simulink model "robot_2015_floor"  (R2017b)
(part 4 of 139)

  Revolute21 : sm_lib/Joints/Revolute Joint  SenseConstraintForce=off  SenseConstraintForceX=off  SenseConstraintForceY=off  SenseConstraintForceZ=off  SenseConstraintTorque=off  SenseConstraintTorqueX=off  SenseConstraintTorqueY=off  SenseConstraintTorqueZ=off  SenseTotalForce=off  SenseTotalForceX=off  SenseTotalForceY=off  SenseTotalForceZ=off  SenseTotalTorque=off  SenseTotalTorqueX=off  SenseTotalTorqueY=off  SenseTotalTorqueZ=off  CompositeWrenchDir=FollowerOnBase  CompositeWrenchFrame=BaseFrame  EquilibriumPosition=0  EquilibriumPositionUnits=rad  SpringStiffness=0  SpringStiffnessUnits=N*m/rad  DampingCoefficient=0  DampingCoefficientUnits=N*m/(rad/s)  TorqueActuationMode=NoTorque  MotionActuationMode=ComputedMotion  SensePosition=off  SenseVelocity=off  SenseAcceleration=off  SenseTorqueForce=off  PositionTargetSpecify=on  PositionTargetPriority=Low  PositionTargetValue=smiData.RevoluteJoint(650).Rz.Pos  PositionTargetValueUnits=deg  VelocityTargetSpecify=off  VelocityTargetPriority=High  VelocityTargetValue=0  VelocityTargetValueUnits=deg/s
  Revolute210 : sm_lib/Joints/Revolute Joint  SenseConstraintForce=off  SenseConstraintForceX=off  SenseConstraintForceY=off  SenseConstraintForceZ=off  SenseConstraintTorque=off  SenseConstraintTorqueX=off  SenseConstraintTorqueY=off  SenseConstraintTorqueZ=off  SenseTotalForce=off  SenseTotalForceX=off  SenseTotalForceY=off  SenseTotalForceZ=off  SenseTotalTorque=off  SenseTotalTorqueX=off  SenseTotalTorqueY=off  SenseTotalTorqueZ=off  CompositeWrenchDir=FollowerOnBase  CompositeWrenchFrame=BaseFrame  EquilibriumPosition=0  EquilibriumPositionUnits=rad  SpringStiffness=0  SpringStiffnessUnits=N*m/rad  DampingCoefficient=0  DampingCoefficientUnits=N*m/(rad/s)  TorqueActuationMode=NoTorque  MotionActuationMode=ComputedMotion  SensePosition=off  SenseVelocity=off  SenseAcceleration=off  SenseTorqueForce=off  PositionTargetSpecify=on  PositionTargetPriority=Low  PositionTargetValue=smiData.RevoluteJoint(839).Rz.Pos  PositionTargetValueUnits=deg  VelocityTargetSpecify=off  VelocityTargetPriority=High  VelocityTargetValue=0  VelocityTargetValueUnits=deg/s
  Revolute211 : sm_lib/Joints/Revolute Joint  SenseConstraintForce=off  SenseConstraintForceX=off  SenseConstraintForceY=off  SenseConstraintForceZ=off  SenseConstraintTorque=off  SenseConstraintTorqueX=off  SenseConstraintTorqueY=off  SenseConstraintTorqueZ=off  SenseTotalForce=off  SenseTotalForceX=off  SenseTotalForceY=off  SenseTotalForceZ=off  SenseTotalTorque=off  SenseTotalTorqueX=off  SenseTotalTorqueY=off  SenseTotalTorqueZ=off  CompositeWrenchDir=FollowerOnBase  CompositeWrenchFrame=BaseFrame  EquilibriumPosition=0  EquilibriumPositionUnits=rad  SpringStiffness=0  SpringStiffnessUnits=N*m/rad  DampingCoefficient=0  DampingCoefficientUnits=N*m/(rad/s)  TorqueActuationMode=NoTorque  MotionActuationMode=ComputedMotion  SensePosition=off  SenseVelocity=off  SenseAcceleration=off  SenseTorqueForce=off  PositionTargetSpecify=on  PositionTargetPriority=Low  PositionTargetValue=smiData.RevoluteJoint(840).Rz.Pos  PositionTargetValueUnits=deg  VelocityTargetSpecify=off  VelocityTargetPriority=High  VelocityTargetValue=0  VelocityTargetValueUnits=deg/s
  Revolute22 : sm_lib/Joints/Revolute Joint  SenseConstraintForce=off  SenseConstraintForceX=off  SenseConstraintForceY=off  SenseConstraintForceZ=off  SenseConstraintTorque=off  SenseConstraintTorqueX=off  SenseConstraintTorqueY=off  SenseConstraintTorqueZ=off  SenseTotalForce=off  SenseTotalForceX=off  SenseTotalForceY=off  SenseTotalForceZ=off  SenseTotalTorque=off  SenseTotalTorqueX=off  SenseTotalTorqueY=off  SenseTotalTorqueZ=off  CompositeWrenchDir=FollowerOnBase  CompositeWrenchFrame=BaseFrame  EquilibriumPosition=0  EquilibriumPositionUnits=rad  SpringStiffness=0  SpringStiffnessUnits=N*m/rad  DampingCoefficient=0  DampingCoefficientUnits=N*m/(rad/s)  TorqueActuationMode=NoTorque  MotionActuationMode=ComputedMotion  SensePosition=off  SenseVelocity=off  SenseAcceleration=off  SenseTorqueForce=off  PositionTargetSpecify=on  PositionTargetPriority=Low  PositionTargetValue=smiData.RevoluteJoint(651).Rz.Pos  PositionTargetValueUnits=deg  VelocityTargetSpecify=off  VelocityTargetPriority=High  VelocityTargetValue=0  VelocityTargetValueUnits=deg/s
  Revolute23 : sm_lib/Joints/Revolute Joint  SenseConstraintForce=off  SenseConstraintForceX=off  SenseConstraintForceY=off  SenseConstraintForceZ=off  SenseConstraintTorque=off  SenseConstraintTorqueX=off  SenseConstraintTorqueY=off  SenseConstraintTorqueZ=off  SenseTotalForce=off  SenseTotalForceX=off  SenseTotalForceY=off  SenseTotalForceZ=off  SenseTotalTorque=off  SenseTotalTorqueX=off  SenseTotalTorqueY=off  SenseTotalTorqueZ=off  CompositeWrenchDir=FollowerOnBase  CompositeWrenchFrame=BaseFrame  EquilibriumPosition=0  EquilibriumPositionUnits=rad  SpringStiffness=0  SpringStiffnessUnits=N*m/rad  DampingCoefficient=0  DampingCoefficientUnits=N*m/(rad/s)  TorqueActuationMode=NoTorque  MotionActuationMode=ComputedMotion  SensePosition=off  SenseVelocity=off  SenseAcceleration=off  SenseTorqueForce=off  PositionTargetSpecify=on  PositionTargetPriority=Low  PositionTargetValue=smiData.RevoluteJoint(652).Rz.Pos  PositionTargetValueUnits=deg  VelocityTargetSpecify=off  VelocityTargetPriority=High  VelocityTargetValue=0  VelocityTargetValueUnits=deg/s
  Revolute24 : sm_lib/Joints/Revolute Joint  SenseConstraintForce=off  SenseConstraintForceX=off  SenseConstraintForceY=off  SenseConstraintForceZ=off  SenseConstraintTorque=off  SenseConstraintTorqueX=off  SenseConstraintTorqueY=off  SenseConstraintTorqueZ=off  SenseTotalForce=off  SenseTotalForceX=off  SenseTotalForceY=off  SenseTotalForceZ=off  SenseTotalTorque=off  SenseTotalTorqueX=off  SenseTotalTorqueY=off  SenseTotalTorqueZ=off  CompositeWrenchDir=FollowerOnBase  CompositeWrenchFrame=BaseFrame  EquilibriumPosition=0  EquilibriumPositionUnits=rad  SpringStiffness=0  SpringStiffnessUnits=N*m/rad  DampingCoefficient=0  DampingCoefficientUnits=N*m/(rad/s)  TorqueActuationMode=NoTorque  MotionActuationMode=ComputedMotion  SensePosition=off  SenseVelocity=off  SenseAcceleration=off  SenseTorqueForce=off  PositionTargetSpecify=on  PositionTargetPriority=Low  PositionTargetValue=smiData.RevoluteJoint(653).Rz.Pos  PositionTargetValueUnits=deg  VelocityTargetSpecify=off  VelocityTargetPriority=High  VelocityTargetValue=0  VelocityTargetValueUnits=deg/s
  Revolute25 : sm_lib/Joints/Revolute Joint  SenseConstraintForce=off  SenseConstraintForceX=off  SenseConstraintForceY=off  SenseConstraintForceZ=off  SenseConstraintTorque=off  SenseConstraintTorqueX=off  SenseConstraintTorqueY=off  SenseConstraintTorqueZ=off  SenseTotalForce=off  SenseTotalForceX=off  SenseTotalForceY=off  SenseTotalForceZ=off  SenseTotalTorque=off  SenseTotalTorqueX=off  SenseTotalTorqueY=off  SenseTotalTorqueZ=off  CompositeWrenchDir=FollowerOnBase  CompositeWrenchFrame=BaseFrame  EquilibriumPosition=0  EquilibriumPositionUnits=rad  SpringStiffness=0  SpringStiffnessUnits=N*m/rad  DampingCoefficient=0  DampingCoefficientUnits=N*m/(rad/s)  TorqueActuationMode=NoTorque  MotionActuationMode=ComputedMotion  SensePosition=off  SenseVelocity=off  SenseAcceleration=off  SenseTorqueForce=off  PositionTargetSpecify=on  PositionTargetPriority=Low  PositionTargetValue=smiData.RevoluteJoint(654).Rz.Pos  PositionTargetValueUnits=deg  VelocityTargetSpecify=off  VelocityTargetPriority=High  VelocityTargetValue=0  VelocityTargetValueUnits=deg/s
  Revolute26 : sm_lib/Joints/Revolute Joint  SenseConstraintForce=off  SenseConstraintForceX=off  SenseConstraintForceY=off  SenseConstraintForceZ=off  SenseConstraintTorque=off  SenseConstraintTorqueX=off  SenseConstraintTorqueY=off  SenseConstraintTorqueZ=off  SenseTotalForce=off  SenseTotalForceX=off  SenseTotalForceY=off  SenseTotalForceZ=off  SenseTotalTorque=off  SenseTotalTorqueX=off  SenseTotalTorqueY=off  SenseTotalTorqueZ=off  CompositeWrenchDir=FollowerOnBase  CompositeWrenchFrame=BaseFrame  EquilibriumPosition=0  EquilibriumPositionUnits=rad  SpringStiffness=0  SpringStiffnessUnits=N*m/rad  DampingCoefficient=0  DampingCoefficientUnits=N*m/(rad/s)  TorqueActuationMode=NoTorque  MotionActuationMode=ComputedMotion  SensePosition=off  SenseVelocity=off  SenseAcceleration=off  SenseTorqueForce=off  PositionTargetSpecify=on  PositionTargetPriority=Low  PositionTargetValue=smiData.RevoluteJoint(655).Rz.Pos  PositionTargetValueUnits=deg  VelocityTargetSpecify=off  VelocityTargetPriority=High  VelocityTargetValue=0  VelocityTargetValueUnits=deg/s
  Revolute27 : sm_lib/Joints/Revolute Joint  SenseConstraintForce=off  SenseConstraintForceX=off  SenseConstraintForceY=off  SenseConstraintForceZ=off  SenseConstraintTorque=off  SenseConstraintTorqueX=off  SenseConstraintTorqueY=off  SenseConstraintTorqueZ=off  SenseTotalForce=off  SenseTotalForceX=off  SenseTotalForceY=off  SenseTotalForceZ=off  SenseTotalTorque=off  SenseTotalTorqueX=off  SenseTotalTorqueY=off  SenseTotalTorqueZ=off  CompositeWrenchDir=FollowerOnBase  CompositeWrenchFrame=BaseFrame  EquilibriumPosition=0  EquilibriumPositionUnits=rad  SpringStiffness=0  SpringStiffnessUnits=N*m/rad  DampingCoefficient=0  DampingCoefficientUnits=N*m/(rad/s)  TorqueActuationMode=NoTorque  MotionActuationMode=ComputedMotion  SensePosition=off  SenseVelocity=off  SenseAcceleration=off  SenseTorqueForce=off  PositionTargetSpecify=on  PositionTargetPriority=Low  PositionTargetValue=smiData.RevoluteJoint(656).Rz.Pos  PositionTargetValueUnits=deg  VelocityTargetSpecify=off  VelocityTargetPriority=High  VelocityTargetValue=0  VelocityTargetValueUnits=deg/s
  Revolute28 : sm_lib/Joints/Revolute Joint  SenseConstraintForce=off  SenseConstraintForceX=off  SenseConstraintForceY=off  SenseConstraintForceZ=off  SenseConstraintTorque=off  SenseConstraintTorqueX=off  SenseConstraintTorqueY=off  SenseConstraintTorqueZ=off  SenseTotalForce=off  SenseTotalForceX=off  SenseTotalForceY=off  SenseTotalForceZ=off  SenseTotalTorque=off  SenseTotalTorqueX=off  SenseTotalTorqueY=off  SenseTotalTorqueZ=off  CompositeWrenchDir=FollowerOnBase  CompositeWrenchFrame=BaseFrame  EquilibriumPosition=0  EquilibriumPositionUnits=rad  SpringStiffness=0  SpringStiffnessUnits=N*m/rad  DampingCoefficient=0  DampingCoefficientUnits=N*m/(rad/s)  TorqueActuationMode=NoTorque  MotionActuationMode=ComputedMotion  SensePosition=off  SenseVelocity=off  SenseAcceleration=off  SenseTorqueForce=off  PositionTargetSpecify=on  PositionTargetPriority=Low  PositionTargetValue=smiData.RevoluteJoint(657).Rz.Pos  PositionTargetValueUnits=deg  VelocityTargetSpecify=off  VelocityTargetPriority=High  VelocityTargetValue=0  VelocityTargetValueUnits=deg/s
  Revolute29 : sm_lib/Joints/Revolute Joint  SenseConstraintForce=off  SenseConstraintForceX=off  SenseConstraintForceY=off  SenseConstraintForceZ=off  SenseConstraintTorque=off  SenseConstraintTorqueX=off  SenseConstraintTorqueY=off  SenseConstraintTorqueZ=off  SenseTotalForce=off  SenseTotalForceX=off  SenseTotalForceY=off  SenseTotalForceZ=off  SenseTotalTorque=off  SenseTotalTorqueX=off  SenseTotalTorqueY=off  SenseTotalTorqueZ=off  CompositeWrenchDir=FollowerOnBase  CompositeWrenchFrame=BaseFrame  EquilibriumPosition=0  EquilibriumPositionUnits=rad  SpringStiffness=0  SpringStiffnessUnits=N*m/rad  DampingCoefficient=0  DampingCoefficientUnits=N*m/(rad/s)  TorqueActuationMode=NoTorque  MotionActuationMode=ComputedMotion  SensePosition=off  SenseVelocity=off  SenseAcceleration=off  SenseTorqueForce=off  PositionTargetSpecify=on  PositionTargetPriority=Low  PositionTargetValue=smiData.RevoluteJoint(658).Rz.Pos  PositionTargetValueUnits=deg  VelocityTargetSpecify=off  VelocityTargetPriority=High  VelocityTargetValue=0  VelocityTargetValueUnits=deg/s
  Revolute3 : sm_lib/Joints/Revolute Joint  SenseConstraintForce=off  SenseConstraintForceX=off  SenseConstraintForceY=off  SenseConstraintForceZ=off  SenseConstraintTorque=off  SenseConstraintTorqueX=off  SenseConstraintTorqueY=off  SenseConstraintTorqueZ=off  SenseTotalForce=off  SenseTotalForceX=off  SenseTotalForceY=off  SenseTotalForceZ=off  SenseTotalTorque=off  SenseTotalTorqueX=off  SenseTotalTorqueY=off  SenseTotalTorqueZ=off  CompositeWrenchDir=FollowerOnBase  CompositeWrenchFrame=BaseFrame  EquilibriumPosition=0  EquilibriumPositionUnits=rad  SpringStiffness=0  SpringStiffnessUnits=N*m/rad  DampingCoefficient=0  DampingCoefficientUnits=N*m/(rad/s)  TorqueActuationMode=NoTorque  MotionActuationMode=ComputedMotion  SensePosition=off  SenseVelocity=off  SenseAcceleration=off  SenseTorqueForce=off  PositionTargetSpecify=on  PositionTargetPriority=Low  PositionTargetValue=smiData.RevoluteJoint(632).Rz.Pos  PositionTargetValueUnits=deg  VelocityTargetSpecify=off  VelocityTargetPriority=High  VelocityTargetValue=0  VelocityTargetValueUnits=deg/s
  Revolute30 : sm_lib/Joints/Revolute Joint  SenseConstraintForce=off  SenseConstraintForceX=off  SenseConstraintForceY=off  SenseConstraintForceZ=off  SenseConstraintTorque=off  SenseConstraintTorqueX=off  SenseConstraintTorqueY=off  SenseConstraintTorqueZ=off  SenseTotalForce=off  SenseTotalForceX=off  SenseTotalForceY=off  SenseTotalForceZ=off  SenseTotalTorque=off  SenseTotalTorqueX=off  SenseTotalTorqueY=off  SenseTotalTorqueZ=off  CompositeWrenchDir=FollowerOnBase  CompositeWrenchFrame=BaseFrame  EquilibriumPosition=0  EquilibriumPositionUnits=rad  SpringStiffness=0  SpringStiffnessUnits=N*m/rad  DampingCoefficient=0  DampingCoefficientUnits=N*m/(rad/s)  TorqueActuationMode=NoTorque  MotionActuationMode=ComputedMotion  SensePosition=off  SenseVelocity=off  SenseAcceleration=off  SenseTorqueForce=off  PositionTargetSpecify=on  PositionTargetPriority=Low  PositionTargetValue=smiData.RevoluteJoint(659).Rz.Pos  PositionTargetValueUnits=deg  VelocityTargetSpecify=off  VelocityTargetPriority=High  VelocityTargetValue=0  VelocityTargetValueUnits=deg/s
  Revolute31 : sm_lib/Joints/Revolute Joint  SenseConstraintForce=off  SenseConstraintForceX=off  SenseConstraintForceY=off  SenseConstraintForceZ=off  SenseConstraintTorque=off  SenseConstraintTorqueX=off  SenseConstraintTorqueY=off  SenseConstraintTorqueZ=off  SenseTotalForce=off  SenseTotalForceX=off  SenseTotalForceY=off  SenseTotalForceZ=off  SenseTotalTorque=off  SenseTotalTorqueX=off  SenseTotalTorqueY=off  SenseTotalTorqueZ=off  CompositeWrenchDir=FollowerOnBase  CompositeWrenchFrame=BaseFrame  EquilibriumPosition=0  EquilibriumPositionUnits=rad  SpringStiffness=0  SpringStiffnessUnits=N*m/rad  DampingCoefficient=0  DampingCoefficientUnits=N*m/(rad/s)  TorqueActuationMode=NoTorque  MotionActuationMode=ComputedMotion  SensePosition=off  SenseVelocity=off  SenseAcceleration=off  SenseTorqueForce=off  PositionTargetSpecify=on  PositionTargetPriority=Low  PositionTargetValue=smiData.RevoluteJoint(660).Rz.Pos  PositionTargetValueUnits=deg  VelocityTargetSpecify=off  VelocityTargetPriority=High  VelocityTargetValue=0  VelocityTargetValueUnits=deg/s
  Revolute32 : sm_lib/Joints/Revolute Joint  SenseConstraintForce=off  SenseConstraintForceX=off  SenseConstraintForceY=off  SenseConstraintForceZ=off  SenseConstraintTorque=off  SenseConstraintTorqueX=off  SenseConstraintTorqueY=off  SenseConstraintTorqueZ=off  SenseTotalForce=off  SenseTotalForceX=off  SenseTotalForceY=off  SenseTotalForceZ=off  SenseTotalTorque=off  SenseTotalTorqueX=off  SenseTotalTorqueY=off  SenseTotalTorqueZ=off  CompositeWrenchDir=FollowerOnBase  CompositeWrenchFrame=BaseFrame  EquilibriumPosition=0  EquilibriumPositionUnits=rad  SpringStiffness=0  SpringStiffnessUnits=N*m/rad  DampingCoefficient=0  DampingCoefficientUnits=N*m/(rad/s)  TorqueActuationMode=NoTorque  MotionActuationMode=ComputedMotion  SensePosition=off  SenseVelocity=off  SenseAcceleration=off  SenseTorqueForce=off  PositionTargetSpecify=on  PositionTargetPriority=Low  PositionTargetValue=smiData.RevoluteJoint(661).Rz.Pos  PositionTargetValueUnits=deg  VelocityTargetSpecify=off  VelocityTargetPriority=High  VelocityTargetValue=0  VelocityTargetValueUnits=deg/s
  Revolute33 : sm_lib/Joints/Revolute Joint  SenseConstraintForce=off  SenseConstraintForceX=off  SenseConstraintForceY=off  SenseConstraintForceZ=off  SenseConstraintTorque=off  SenseConstraintTorqueX=off  SenseConstraintTorqueY=off  SenseConstraintTorqueZ=off  SenseTotalForce=off  SenseTotalForceX=off  SenseTotalForceY=off  SenseTotalForceZ=off  SenseTotalTorque=off  SenseTotalTorqueX=off  SenseTotalTorqueY=off  SenseTotalTorqueZ=off  CompositeWrenchDir=FollowerOnBase  CompositeWrenchFrame=BaseFrame  EquilibriumPosition=0  EquilibriumPositionUnits=rad  SpringStiffness=0  SpringStiffnessUnits=N*m/rad  DampingCoefficient=0  DampingCoefficientUnits=N*m/(rad/s)  TorqueActuationMode=NoTorque  MotionActuationMode=ComputedMotion  SensePosition=off  SenseVelocity=off  SenseAcceleration=off  SenseTorqueForce=off  PositionTargetSpecify=on  PositionTargetPriority=Low  PositionTargetValue=smiData.RevoluteJoint(662).Rz.Pos  PositionTargetValueUnits=deg  VelocityTargetSpecify=off  VelocityTargetPriority=High  VelocityTargetValue=0  VelocityTargetValueUnits=deg/s
  Revolute34 : sm_lib/Joints/Revolute Joint  SenseConstraintForce=off  SenseConstraintForceX=off  SenseConstraintForceY=off  SenseConstraintForceZ=off  SenseConstraintTorque=off  SenseConstraintTorqueX=off  SenseConstraintTorqueY=off  SenseConstraintTorqueZ=off  SenseTotalForce=off  SenseTotalForceX=off  SenseTotalForceY=off  SenseTotalForceZ=off  SenseTotalTorque=off  SenseTotalTorqueX=off  SenseTotalTorqueY=off  SenseTotalTorqueZ=off  CompositeWrenchDir=FollowerOnBase  CompositeWrenchFrame=BaseFrame  EquilibriumPosition=0  EquilibriumPositionUnits=rad  SpringStiffness=0  SpringStiffnessUnits=N*m/rad  DampingCoefficient=0  DampingCoefficientUnits=N*m/(rad/s)  TorqueActuationMode=NoTorque  MotionActuationMode=ComputedMotion  SensePosition=off  SenseVelocity=off  SenseAcceleration=off  SenseTorqueForce=off  PositionTargetSpecify=on  PositionTargetPriority=Low  PositionTargetValue=smiData.RevoluteJoint(663).Rz.Pos  PositionTargetValueUnits=deg  VelocityTargetSpecify=off  VelocityTargetPriority=High  VelocityTargetValue=0  VelocityTargetValueUnits=deg/s
  Revolute35 : sm_lib/Joints/Revolute Joint  SenseConstraintForce=off  SenseConstraintForceX=off  SenseConstraintForceY=off  SenseConstraintForceZ=off  SenseConstraintTorque=off  SenseConstraintTorqueX=off  SenseConstraintTorqueY=off  SenseConstraintTorqueZ=off  SenseTotalForce=off  SenseTotalForceX=off  SenseTotalForceY=off  SenseTotalForceZ=off  SenseTotalTorque=off  SenseTotalTorqueX=off  SenseTotalTorqueY=off  SenseTotalTorqueZ=off  CompositeWrenchDir=FollowerOnBase  CompositeWrenchFrame=BaseFrame  EquilibriumPosition=0  EquilibriumPositionUnits=rad  SpringStiffness=0  SpringStiffnessUnits=N*m/rad  DampingCoefficient=0  DampingCoefficientUnits=N*m/(rad/s)  TorqueActuationMode=NoTorque  MotionActuationMode=ComputedMotion  SensePosition=off  SenseVelocity=off  SenseAcceleration=off  SenseTorqueForce=off  PositionTargetSpecify=on  PositionTargetPriority=Low  PositionTargetValue=smiData.RevoluteJoint(664).Rz.Pos  PositionTargetValueUnits=deg  VelocityTargetSpecify=off  VelocityTargetPriority=High  VelocityTargetValue=0  VelocityTargetValueUnits=deg/s
  Revolute36 : sm_lib/Joints/Revolute Joint  SenseConstraintForce=off  SenseConstraintForceX=off  SenseConstraintForceY=off  SenseConstraintForceZ=off  SenseConstraintTorque=off  SenseConstraintTorqueX=off  SenseConstraintTorqueY=off  SenseConstraintTorqueZ=off  SenseTotalForce=off  SenseTotalForceX=off  SenseTotalForceY=off  SenseTotalForceZ=off  SenseTotalTorque=off  SenseTotalTorqueX=off  SenseTotalTorqueY=off  SenseTotalTorqueZ=off  CompositeWrenchDir=FollowerOnBase  CompositeWrenchFrame=BaseFrame  EquilibriumPosition=0  EquilibriumPositionUnits=rad  SpringStiffness=0  SpringStiffnessUnits=N*m/rad  DampingCoefficient=0  DampingCoefficientUnits=N*m/(rad/s)  TorqueActuationMode=NoTorque  MotionActuationMode=ComputedMotion  SensePosition=off  SenseVelocity=off  SenseAcceleration=off  SenseTorqueForce=off  PositionTargetSpecify=on  PositionTargetPriority=Low  PositionTargetValue=smiData.RevoluteJoint(665).Rz.Pos  PositionTargetValueUnits=deg  VelocityTargetSpecify=off  VelocityTargetPriority=High  VelocityTargetValue=0  VelocityTargetValueUnits=deg/s
  Revolute37 : sm_lib/Joints/Revolute Joint  SenseConstraintForce=off  SenseConstraintForceX=off  SenseConstraintForceY=off  SenseConstraintForceZ=off  SenseConstraintTorque=off  SenseConstraintTorqueX=off  SenseConstraintTorqueY=off  SenseConstraintTorqueZ=off  SenseTotalForce=off  SenseTotalForceX=off  SenseTotalForceY=off  SenseTotalForceZ=off  SenseTotalTorque=off  SenseTotalTorqueX=off  SenseTotalTorqueY=off  SenseTotalTorqueZ=off  CompositeWrenchDir=FollowerOnBase  CompositeWrenchFrame=BaseFrame  EquilibriumPosition=0  EquilibriumPositionUnits=rad  SpringStiffness=0  SpringStiffnessUnits=N*m/rad  DampingCoefficient=0  DampingCoefficientUnits=N*m/(rad/s)  TorqueActuationMode=NoTorque  MotionActuationMode=ComputedMotion  SensePosition=off  SenseVelocity=off  SenseAcceleration=off  SenseTorqueForce=off  PositionTargetSpecify=on  PositionTargetPriority=Low  PositionTargetValue=smiData.RevoluteJoint(666).Rz.Pos  PositionTargetValueUnits=deg  VelocityTargetSpecify=off  VelocityTargetPriority=High  VelocityTargetValue=0  VelocityTargetValueUnits=deg/s
  Revolute38 : sm_lib/Joints/Revolute Joint  SenseConstraintForce=off  SenseConstraintForceX=off  SenseConstraintForceY=off  SenseConstraintForceZ=off  SenseConstraintTorque=off  SenseConstraintTorqueX=off  SenseConstraintTorqueY=off  SenseConstraintTorqueZ=off  SenseTotalForce=off  SenseTotalForceX=off  SenseTotalForceY=off  SenseTotalForceZ=off  SenseTotalTorque=off  SenseTotalTorqueX=off  SenseTotalTorqueY=off  SenseTotalTorqueZ=off  CompositeWrenchDir=FollowerOnBase  CompositeWrenchFrame=BaseFrame  EquilibriumPosition=0  EquilibriumPositionUnits=rad  SpringStiffness=0  SpringStiffnessUnits=N*m/rad  DampingCoefficient=0  DampingCoefficientUnits=N*m/(rad/s)  TorqueActuationMode=NoTorque  MotionActuationMode=ComputedMotion  SensePosition=off  SenseVelocity=off  SenseAcceleration=off  SenseTorqueForce=off  PositionTargetSpecify=on  PositionTargetPriority=Low  PositionTargetValue=smiData.RevoluteJoint(667).Rz.Pos  PositionTargetValueUnits=deg  VelocityTargetSpecify=off  VelocityTargetPriority=High  VelocityTargetValue=0  VelocityTargetValueUnits=deg/s
  Revolute39 : sm_lib/Joints/Revolute Joint  SenseConstraintForce=off  SenseConstraintForceX=off  SenseConstraintForceY=off  SenseConstraintForceZ=off  SenseConstraintTorque=off  SenseConstraintTorqueX=off  SenseConstraintTorqueY=off  SenseConstraintTorqueZ=off  SenseTotalForce=off  SenseTotalForceX=off  SenseTotalForceY=off  SenseTotalForceZ=off  SenseTotalTorque=off  SenseTotalTorqueX=off  SenseTotalTorqueY=off  SenseTotalTorqueZ=off  CompositeWrenchDir=FollowerOnBase  CompositeWrenchFrame=BaseFrame  EquilibriumPosition=0  EquilibriumPositionUnits=rad  SpringStiffness=0  SpringStiffnessUnits=N*m/rad  DampingCoefficient=0  DampingCoefficientUnits=N*m/(rad/s)  TorqueActuationMode=NoTorque  MotionActuationMode=ComputedMotion  SensePosition=off  SenseVelocity=off  SenseAcceleration=off  SenseTorqueForce=off  PositionTargetSpecify=on  PositionTargetPriority=Low  PositionTargetValue=smiData.RevoluteJoint(668).Rz.Pos  PositionTargetValueUnits=deg  VelocityTargetSpecify=off  VelocityTargetPriority=High  VelocityTargetValue=0  VelocityTargetValueUnits=deg/s
  Revolute4 : sm_lib/Joints/Revolute Joint  SenseConstraintForce=off  SenseConstraintForceX=off  SenseConstraintForceY=off  SenseConstraintForceZ=off  SenseConstraintTorque=off  SenseConstraintTorqueX=off  SenseConstraintTorqueY=off  SenseConstraintTorqueZ=off  SenseTotalForce=off  SenseTotalForceX=off  SenseTotalForceY=off  SenseTotalForceZ=off  SenseTotalTorque=off  SenseTotalTorqueX=off  SenseTotalTorqueY=off  SenseTotalTorqueZ=off  CompositeWrenchDir=FollowerOnBase  CompositeWrenchFrame=BaseFrame  EquilibriumPosition=0  EquilibriumPositionUnits=rad  SpringStiffness=0  SpringStiffnessUnits=N*m/rad  DampingCoefficient=0  DampingCoefficientUnits=N*m/(rad/s)  TorqueActuationMode=NoTorque  MotionActuationMode=ComputedMotion  SensePosition=off  SenseVelocity=off  SenseAcceleration=off  SenseTorqueForce=off  PositionTargetSpecify=on  PositionTargetPriority=Low  PositionTargetValue=smiData.RevoluteJoint(633).Rz.Pos  PositionTargetValueUnits=deg  VelocityTargetSpecify=off  VelocityTargetPriority=High  VelocityTargetValue=0  VelocityTargetValueUnits=deg/s
  Revolute40 : sm_lib/Joints/Revolute Joint  SenseConstraintForce=off  SenseConstraintForceX=off  SenseConstraintForceY=off  SenseConstraintForceZ=off  SenseConstraintTorque=off  SenseConstraintTorqueX=off  SenseConstraintTorqueY=off  SenseConstraintTorqueZ=off  SenseTotalForce=off  SenseTotalForceX=off  SenseTotalForceY=off  SenseTotalForceZ=off  SenseTotalTorque=off  SenseTotalTorqueX=off  SenseTotalTorqueY=off  SenseTotalTorqueZ=off  CompositeWrenchDir=FollowerOnBase  CompositeWrenchFrame=BaseFrame  EquilibriumPosition=0  EquilibriumPositionUnits=rad  SpringStiffness=0  SpringStiffnessUnits=N*m/rad  DampingCoefficient=0  DampingCoefficientUnits=N*m/(rad/s)  TorqueActuationMode=NoTorque  MotionActuationMode=ComputedMotion  SensePosition=off  SenseVelocity=off  SenseAcceleration=off  SenseTorqueForce=off  PositionTargetSpecify=on  PositionTargetPriority=Low  PositionTargetValue=smiData.RevoluteJoint(669).Rz.Pos  PositionTargetValueUnits=deg  VelocityTargetSpecify=off  VelocityTargetPriority=High  VelocityTargetValue=0  VelocityTargetValueUnits=deg/s
  Revolute41 : sm_lib/Joints/Revolute Joint  SenseConstraintForce=off  SenseConstraintForceX=off  SenseConstraintForceY=off  SenseConstraintForceZ=off  SenseConstraintTorque=off  SenseConstraintTorqueX=off  SenseConstraintTorqueY=off  SenseConstraintTorqueZ=off  SenseTotalForce=off  SenseTotalForceX=off  SenseTotalForceY=off  SenseTotalForceZ=off  SenseTotalTorque=off  SenseTotalTorqueX=off  SenseTotalTorqueY=off  SenseTotalTorqueZ=off  CompositeWrenchDir=FollowerOnBase  CompositeWrenchFrame=BaseFrame  EquilibriumPosition=0  EquilibriumPositionUnits=rad  SpringStiffness=0  SpringStiffnessUnits=N*m/rad  DampingCoefficient=0  DampingCoefficientUnits=N*m/(rad/s)  TorqueActuationMode=NoTorque  MotionActuationMode=ComputedMotion  SensePosition=off  SenseVelocity=off  SenseAcceleration=off  SenseTorqueForce=off  PositionTargetSpecify=on  PositionTargetPriority=Low  PositionTargetValue=smiData.RevoluteJoint(670).Rz.Pos  PositionTargetValueUnits=deg  VelocityTargetSpecify=off  VelocityTargetPriority=High  VelocityTargetValue=0  VelocityTargetValueUnits=deg/s
  Revolute42 : sm_lib/Joints/Revolute Joint  SenseConstraintForce=off  SenseConstraintForceX=off  SenseConstraintForceY=off  SenseConstraintForceZ=off  SenseConstraintTorque=off  SenseConstraintTorqueX=off  SenseConstraintTorqueY=off  SenseConstraintTorqueZ=off  SenseTotalForce=off  SenseTotalForceX=off  SenseTotalForceY=off  SenseTotalForceZ=off  SenseTotalTorque=off  SenseTotalTorqueX=off  SenseTotalTorqueY=off  SenseTotalTorqueZ=off  CompositeWrenchDir=FollowerOnBase  CompositeWrenchFrame=BaseFrame  EquilibriumPosition=0  EquilibriumPositionUnits=rad  SpringStiffness=0  SpringStiffnessUnits=N*m/rad  DampingCoefficient=0  DampingCoefficientUnits=N*m/(rad/s)  TorqueActuationMode=NoTorque  MotionActuationMode=ComputedMotion  SensePosition=off  SenseVelocity=off  SenseAcceleration=off  SenseTorqueForce=off  PositionTargetSpecify=on  PositionTargetPriority=Low  PositionTargetValue=smiData.RevoluteJoint(671).Rz.Pos  PositionTargetValueUnits=deg  VelocityTargetSpecify=off  VelocityTargetPriority=High  VelocityTargetValue=0  VelocityTargetValueUnits=deg/s
  Revolute43 : sm_lib/Joints/Revolute Joint  SenseConstraintForce=off  SenseConstraintForceX=off  SenseConstraintForceY=off  SenseConstraintForceZ=off  SenseConstraintTorque=off  SenseConstraintTorqueX=off  SenseConstraintTorqueY=off  SenseConstraintTorqueZ=off  SenseTotalForce=off  SenseTotalForceX=off  SenseTotalForceY=off  SenseTotalForceZ=off  SenseTotalTorque=off  SenseTotalTorqueX=off  SenseTotalTorqueY=off  SenseTotalTorqueZ=off  CompositeWrenchDir=FollowerOnBase  CompositeWrenchFrame=BaseFrame  EquilibriumPosition=0  EquilibriumPositionUnits=rad  SpringStiffness=0  SpringStiffnessUnits=N*m/rad  DampingCoefficient=0  DampingCoefficientUnits=N*m/(rad/s)  TorqueActuationMode=NoTorque  MotionActuationMode=ComputedMotion  SensePosition=off  SenseVelocity=off  SenseAcceleration=off  SenseTorqueForce=off  PositionTargetSpecify=on  PositionTargetPriority=Low  PositionTargetValue=smiData.RevoluteJoint(672).Rz.Pos  PositionTargetValueUnits=deg  VelocityTargetSpecify=off  VelocityTargetPriority=High  VelocityTargetValue=0  VelocityTargetValueUnits=deg/s
  Revolute44 : sm_lib/Joints/Revolute Joint  SenseConstraintForce=off  SenseConstraintForceX=off  SenseConstraintForceY=off  SenseConstraintForceZ=off  SenseConstraintTorque=off  SenseConstraintTorqueX=off  SenseConstraintTorqueY=off  SenseConstraintTorqueZ=off  SenseTotalForce=off  SenseTotalForceX=off  SenseTotalForceY=off  SenseTotalForceZ=off  SenseTotalTorque=off  SenseTotalTorqueX=off  SenseTotalTorqueY=off  SenseTotalTorqueZ=off  CompositeWrenchDir=FollowerOnBase  CompositeWrenchFrame=BaseFrame  EquilibriumPosition=0  EquilibriumPositionUnits=rad  SpringStiffness=0  SpringStiffnessUnits=N*m/rad  DampingCoefficient=0  DampingCoefficientUnits=N*m/(rad/s)  TorqueActuationMode=NoTorque  MotionActuationMode=ComputedMotion  SensePosition=off  SenseVelocity=off  SenseAcceleration=off  SenseTorqueForce=off  PositionTargetSpecify=on  PositionTargetPriority=Low  PositionTargetValue=smiData.RevoluteJoint(673).Rz.Pos  PositionTargetValueUnits=deg  VelocityTargetSpecify=off  VelocityTargetPriority=High  VelocityTargetValue=0  VelocityTargetValueUnits=deg/s
  Revolute45 : sm_lib/Joints/Revolute Joint  SenseConstraintForce=off  SenseConstraintForceX=off  SenseConstraintForceY=off  SenseConstraintForceZ=off  SenseConstraintTorque=off  SenseConstraintTorqueX=off  SenseConstraintTorqueY=off  SenseConstraintTorqueZ=off  SenseTotalForce=off  SenseTotalForceX=off  SenseTotalForceY=off  SenseTotalForceZ=off  SenseTotalTorque=off  SenseTotalTorqueX=off  SenseTotalTorqueY=off  SenseTotalTorqueZ=off  CompositeWrenchDir=FollowerOnBase  CompositeWrenchFrame=BaseFrame  EquilibriumPosition=0  EquilibriumPositionUnits=rad  SpringStiffness=0  SpringStiffnessUnits=N*m/rad  DampingCoefficient=0  DampingCoefficientUnits=N*m/(rad/s)  TorqueActuationMode=NoTorque  MotionActuationMode=ComputedMotion  SensePosition=off  SenseVelocity=off  SenseAcceleration=off  SenseTorqueForce=off  PositionTargetSpecify=off  PositionTargetPriority=High  PositionTargetValue=0  PositionTargetValueUnits=deg  VelocityTargetSpecify=off  VelocityTargetPriority=High  VelocityTargetValue=0  VelocityTargetValueUnits=deg/s
  Revolute46 : sm_lib/Joints/Revolute Joint  SenseConstraintForce=off  SenseConstraintForceX=off  SenseConstraintForceY=off  SenseConstraintForceZ=off  SenseConstraintTorque=off  SenseConstraintTorqueX=off  SenseConstraintTorqueY=off  SenseConstraintTorqueZ=off  SenseTotalForce=off  SenseTotalForceX=off  SenseTotalForceY=off  SenseTotalForceZ=off  SenseTotalTorque=off  SenseTotalTorqueX=off  SenseTotalTorqueY=off  SenseTotalTorqueZ=off  CompositeWrenchDir=FollowerOnBase  CompositeWrenchFrame=BaseFrame  EquilibriumPosition=0  EquilibriumPositionUnits=rad  SpringStiffness=0  SpringStiffnessUnits=N*m/rad  DampingCoefficient=0  DampingCoefficientUnits=N*m/(rad/s)  TorqueActuationMode=NoTorque  MotionActuationMode=ComputedMotion  SensePosition=off  SenseVelocity=off  SenseAcceleration=off  SenseTorqueForce=off  PositionTargetSpecify=on  PositionTargetPriority=Low  PositionTargetValue=smiData.RevoluteJoint(675).Rz.Pos  PositionTargetValueUnits=deg  VelocityTargetSpecify=off  VelocityTargetPriority=High  VelocityTargetValue=0  VelocityTargetValueUnits=deg/s
  Revolute47 : sm_lib/Joints/Revolute Joint  SenseConstraintForce=off  SenseConstraintForceX=off  SenseConstraintForceY=off  SenseConstraintForceZ=off  SenseConstraintTorque=off  SenseConstraintTorqueX=off  SenseConstraintTorqueY=off  SenseConstraintTorqueZ=off  SenseTotalForce=off  SenseTotalForceX=off  SenseTotalForceY=off  SenseTotalForceZ=off  SenseTotalTorque=off  SenseTotalTorqueX=off  SenseTotalTorqueY=off  SenseTotalTorqueZ=off  CompositeWrenchDir=FollowerOnBase  CompositeWrenchFrame=BaseFrame  EquilibriumPosition=0  EquilibriumPositionUnits=rad  SpringStiffness=0  SpringStiffnessUnits=N*m/rad  DampingCoefficient=0  DampingCoefficientUnits=N*m/(rad/s)  TorqueActuationMode=InputTorque  MotionActuationMode=ComputedMotion  SensePosition=on  SenseVelocity=on  SenseAcceleration=off  SenseTorqueForce=off  PositionTargetSpecify=on  PositionTargetPriority=High  PositionTargetValue=3.14  PositionTargetValueUnits=rad  VelocityTargetSpecify=off  VelocityTargetPriority=High  VelocityTargetValue=0  VelocityTargetValueUnits=deg/s
  Revolute48 : sm_lib/Joints/Revolute Joint  SenseConstraintForce=off  SenseConstraintForceX=off  SenseConstraintForceY=off  SenseConstraintForceZ=off  SenseConstraintTorque=off  SenseConstraintTorqueX=off  SenseConstraintTorqueY=off  SenseConstraintTorqueZ=off  SenseTotalForce=off  SenseTotalForceX=off  SenseTotalForceY=off  SenseTotalForceZ=off  SenseTotalTorque=off  SenseTotalTorqueX=off  SenseTotalTorqueY=off  SenseTotalTorqueZ=off  CompositeWrenchDir=FollowerOnBase  CompositeWrenchFrame=BaseFrame  EquilibriumPosition=0  EquilibriumPositionUnits=rad  SpringStiffness=0  SpringStiffnessUnits=N*m/rad  DampingCoefficient=0  DampingCoefficientUnits=N*m/(rad/s)  TorqueActuationMode=InputTorque  MotionActuationMode=ComputedMotion  SensePosition=on  SenseVelocity=on  SenseAcceleration=off  SenseTorqueForce=off  PositionTargetSpecify=on  PositionTargetPriority=High  PositionTargetValue=-1  PositionTargetValueUnits=rad  VelocityTargetSpecify=off  VelocityTargetPriority=High  VelocityTargetValue=0  VelocityTargetValueUnits=deg/s
  Revolute49 : sm_lib/Joints/Revolute Joint  SenseConstraintForce=off  SenseConstraintForceX=off  SenseConstraintForceY=off  SenseConstraintForceZ=off  SenseConstraintTorque=off  SenseConstraintTorqueX=off  SenseConstraintTorqueY=off  SenseConstraintTorqueZ=off  SenseTotalForce=off  SenseTotalForceX=off  SenseTotalForceY=off  SenseTotalForceZ=off  SenseTotalTorque=off  SenseTotalTorqueX=off  SenseTotalTorqueY=off  SenseTotalTorqueZ=off  CompositeWrenchDir=FollowerOnBase  CompositeWrenchFrame=BaseFrame  EquilibriumPosition=0  EquilibriumPositionUnits=rad  SpringStiffness=0  SpringStiffnessUnits=N*m/rad  DampingCoefficient=0  DampingCoefficientUnits=N*m/(rad/s)  TorqueActuationMode=InputTorque  MotionActuationMode=ComputedMotion  SensePosition=on  SenseVelocity=on  SenseAcceleration=off  SenseTorqueForce=off  PositionTargetSpecify=on  PositionTargetPriority=High  PositionTargetValue=1.57  PositionTargetValueUnits=rad  VelocityTargetSpecify=off  VelocityTargetPriority=High  VelocityTargetValue=0  VelocityTargetValueUnits=deg/s
  Revolute5 : sm_lib/Joints/Revolute Joint  SenseConstraintForce=off  SenseConstraintForceX=off  SenseConstraintForceY=off  SenseConstraintForceZ=off  SenseConstraintTorque=off  SenseConstraintTorqueX=off  SenseConstraintTorqueY=off  SenseConstraintTorqueZ=off  SenseTotalForce=off  SenseTotalForceX=off  SenseTotalForceY=off  SenseTotalForceZ=off  SenseTotalTorque=off  SenseTotalTorqueX=off  SenseTotalTorqueY=off  SenseTotalTorqueZ=off  CompositeWrenchDir=FollowerOnBase  CompositeWrenchFrame=BaseFrame  EquilibriumPosition=0  EquilibriumPositionUnits=rad  SpringStiffness=0  SpringStiffnessUnits=N*m/rad  DampingCoefficient=0  DampingCoefficientUnits=N*m/(rad/s)  TorqueActuationMode=NoTorque  MotionActuationMode=ComputedMotion  SensePosition=off  SenseVelocity=off  SenseAcceleration=off  SenseTorqueForce=off  PositionTargetSpecify=on  PositionTargetPriority=Low  PositionTargetValue=smiData.RevoluteJoint(634).Rz.Pos  PositionTargetValueUnits=deg  VelocityTargetSpecify=off  VelocityTargetPriority=High  VelocityTargetValue=0  VelocityTargetValueUnits=deg/s
  Revolute50 : sm_lib/Joints/Revolute Joint  SenseConstraintForce=off  SenseConstraintForceX=off  SenseConstraintForceY=off  SenseConstraintForceZ=off  SenseConstraintTorque=off  SenseConstraintTorqueX=off  SenseConstraintTorqueY=off  SenseConstraintTorqueZ=off  SenseTotalForce=off  SenseTotalForceX=off  SenseTotalForceY=off  SenseTotalForceZ=off  SenseTotalTorque=off  SenseTotalTorqueX=off  SenseTotalTorqueY=off  SenseTotalTorqueZ=off  CompositeWrenchDir=FollowerOnBase  CompositeWrenchFrame=BaseFrame  EquilibriumPosition=0  EquilibriumPositionUnits=rad  SpringStiffness=0  SpringStiffnessUnits=N*m/rad  DampingCoefficient=0  DampingCoefficientUnits=N*m/(rad/s)  TorqueActuationMode=NoTorque  MotionActuationMode=ComputedMotion  SensePosition=off  SenseVelocity=off  SenseAcceleration=off  SenseTorqueForce=off  PositionTargetSpecify=on  PositionTargetPriority=Low  PositionTargetValue=smiData.RevoluteJoint(679).Rz.Pos  PositionTargetValueUnits=deg  VelocityTargetSpecify=off  VelocityTargetPriority=High  VelocityTargetValue=0  VelocityTargetValueUnits=deg/s
  Revolute51 : sm_lib/Joints/Revolute Joint  SenseConstraintForce=off  SenseConstraintForceX=off  SenseConstraintForceY=off  SenseConstraintForceZ=off  SenseConstraintTorque=off  SenseConstraintTorqueX=off  SenseConstraintTorqueY=off  SenseConstraintTorqueZ=off  SenseTotalForce=off  SenseTotalForceX=off  SenseTotalForceY=off  SenseTotalForceZ=off  SenseTotalTorque=off  SenseTotalTorqueX=off  SenseTotalTorqueY=off  SenseTotalTorqueZ=off  CompositeWrenchDir=FollowerOnBase  CompositeWrenchFrame=BaseFrame  EquilibriumPosition=0  EquilibriumPositionUnits=rad  SpringStiffness=0  SpringStiffnessUnits=N*m/rad  DampingCoefficient=0  DampingCoefficientUnits=N*m/(rad/s)  TorqueActuationMode=NoTorque  MotionActuationMode=ComputedMotion  SensePosition=off  SenseVelocity=off  SenseAcceleration=off  SenseTorqueForce=off  PositionTargetSpecify=on  PositionTargetPriority=Low  PositionTargetValue=smiData.RevoluteJoint(680).Rz.Pos  PositionTargetValueUnits=deg  VelocityTargetSpecify=off  VelocityTargetPriority=High  VelocityTargetValue=0  VelocityTargetValueUnits=deg/s
  Revolute52 : sm_lib/Joints/Revolute Joint  SenseConstraintForce=off  SenseConstraintForceX=off  SenseConstraintForceY=off  SenseConstraintForceZ=off  SenseConstraintTorque=off  SenseConstraintTorqueX=off  SenseConstraintTorqueY=off  SenseConstraintTorqueZ=off  SenseTotalForce=off  SenseTotalForceX=off  SenseTotalForceY=off  SenseTotalForceZ=off  SenseTotalTorque=off  SenseTotalTorqueX=off  SenseTotalTorqueY=off  SenseTotalTorqueZ=off  CompositeWrenchDir=FollowerOnBase  CompositeWrenchFrame=BaseFrame  EquilibriumPosition=0  EquilibriumPositionUnits=rad  SpringStiffness=0  SpringStiffnessUnits=N*m/rad  DampingCoefficient=0  DampingCoefficientUnits=N*m/(rad/s)  TorqueActuationMode=NoTorque  MotionActuationMode=ComputedMotion  SensePosition=off  SenseVelocity=off  SenseAcceleration=off  SenseTorqueForce=off  PositionTargetSpecify=on  PositionTargetPriority=Low  PositionTargetValue=smiData.RevoluteJoint(681).Rz.Pos  PositionTargetValueUnits=deg  VelocityTargetSpecify=off  VelocityTargetPriority=High  VelocityTargetValue=0  VelocityTargetValueUnits=deg/s
  Revolute53 : sm_lib/Joints/Revolute Joint  SenseConstraintForce=off  SenseConstraintForceX=off  SenseConstraintForceY=off  SenseConstraintForceZ=off  SenseConstraintTorque=off  SenseConstraintTorqueX=off  SenseConstraintTorqueY=off  SenseConstraintTorqueZ=off  SenseTotalForce=off  SenseTotalForceX=off  SenseTotalForceY=off  SenseTotalForceZ=off  SenseTotalTorque=off  SenseTotalTorqueX=off  SenseTotalTorqueY=off  SenseTotalTorqueZ=off  CompositeWrenchDir=FollowerOnBase  CompositeWrenchFrame=BaseFrame  EquilibriumPosition=0  EquilibriumPositionUnits=rad  SpringStiffness=0  SpringStiffnessUnits=N*m/rad  DampingCoefficient=0  DampingCoefficientUnits=N*m/(rad/s)  TorqueActuationMode=NoTorque  MotionActuationMode=ComputedMotion  SensePosition=off  SenseVelocity=off  SenseAcceleration=off  SenseTorqueForce=off  PositionTargetSpecify=on  PositionTargetPriority=Low  PositionTargetValue=smiData.RevoluteJoint(682).Rz.Pos  PositionTargetValueUnits=deg  VelocityTargetSpecify=off  VelocityTargetPriority=High  VelocityTargetValue=0  VelocityTargetValueUnits=deg/s
  Revolute54 : sm_lib/Joints/Revolute Joint  SenseConstraintForce=off  SenseConstraintForceX=off  SenseConstraintForceY=off  SenseConstraintForceZ=off  SenseConstraintTorque=off  SenseConstraintTorqueX=off  SenseConstraintTorqueY=off  SenseConstraintTorqueZ=off  SenseTotalForce=off  SenseTotalForceX=off  SenseTotalForceY=off  SenseTotalForceZ=off  SenseTotalTorque=off  SenseTotalTorqueX=off  SenseTotalTorqueY=off  SenseTotalTorqueZ=off  CompositeWrenchDir=FollowerOnBase  CompositeWrenchFrame=BaseFrame  EquilibriumPosition=0  EquilibriumPositionUnits=rad  SpringStiffness=0  SpringStiffnessUnits=N*m/rad  DampingCoefficient=0  DampingCoefficientUnits=N*m/(rad/s)  TorqueActuationMode=NoTorque  MotionActuationMode=ComputedMotion  SensePosition=off  SenseVelocity=off  SenseAcceleration=off  SenseTorqueForce=off  PositionTargetSpecify=on  PositionTargetPriority=Low  PositionTargetValue=smiData.RevoluteJoint(683).Rz.Pos  PositionTargetValueUnits=deg  VelocityTargetSpecify=off  VelocityTargetPriority=High  VelocityTargetValue=0  VelocityTargetValueUnits=deg/s
  Revolute55 : sm_lib/Joints/Revolute Joint  SenseConstraintForce=off  SenseConstraintForceX=off  SenseConstraintForceY=off  SenseConstraintForceZ=off  SenseConstraintTorque=off  SenseConstraintTorqueX=off  SenseConstraintTorqueY=off  SenseConstraintTorqueZ=off  SenseTotalForce=off  SenseTotalForceX=off  SenseTotalForceY=off  SenseTotalForceZ=off  SenseTotalTorque=off  SenseTotalTorqueX=off  SenseTotalTorqueY=off  SenseTotalTorqueZ=off  CompositeWrenchDir=FollowerOnBase  CompositeWrenchFrame=BaseFrame  EquilibriumPosition=0  EquilibriumPositionUnits=rad  SpringStiffness=0  SpringStiffnessUnits=N*m/rad  DampingCoefficient=0  DampingCoefficientUnits=N*m/(rad/s)  TorqueActuationMode=NoTorque  MotionActuationMode=ComputedMotion  SensePosition=off  SenseVelocity=off  SenseAcceleration=off  SenseTorqueForce=off  PositionTargetSpecify=on  PositionTargetPriority=Low  PositionTargetValue=smiData.RevoluteJoint(684).Rz.Pos  PositionTargetValueUnits=deg  VelocityTargetSpecify=off  VelocityTargetPriority=High  VelocityTargetValue=0  VelocityTargetValueUnits=deg/s
  Revolute56 : sm_lib/Joints/Revolute Joint  SenseConstraintForce=off  SenseConstraintForceX=off  SenseConstraintForceY=off  SenseConstraintForceZ=off  SenseConstraintTorque=off  SenseConstraintTorqueX=off  SenseConstraintTorqueY=off  SenseConstraintTorqueZ=off  SenseTotalForce=off  SenseTotalForceX=off  SenseTotalForceY=off  SenseTotalForceZ=off  SenseTotalTorque=off  SenseTotalTorqueX=off  SenseTotalTorqueY=off  SenseTotalTorqueZ=off  CompositeWrenchDir=FollowerOnBase  CompositeWrenchFrame=BaseFrame  EquilibriumPosition=0  EquilibriumPositionUnits=rad  SpringStiffness=0  SpringStiffnessUnits=N*m/rad  DampingCoefficient=0  DampingCoefficientUnits=N*m/(rad/s)  TorqueActuationMode=NoTorque  MotionActuationMode=ComputedMotion  SensePosition=off  SenseVelocity=off  SenseAcceleration=off  SenseTorqueForce=off  PositionTargetSpecify=on  PositionTargetPriority=Low  PositionTargetValue=smiData.RevoluteJoint(685).Rz.Pos  PositionTargetValueUnits=deg  VelocityTargetSpecify=off  VelocityTargetPriority=High  VelocityTargetValue=0  VelocityTargetValueUnits=deg/s
  Revolute57 : sm_lib/Joints/Revolute Joint  SenseConstraintForce=off  SenseConstraintForceX=off  SenseConstraintForceY=off  SenseConstraintForceZ=off  SenseConstraintTorque=off  SenseConstraintTorqueX=off  SenseConstraintTorqueY=off  SenseConstraintTorqueZ=off  SenseTotalForce=off  SenseTotalForceX=off  SenseTotalForceY=off  SenseTotalForceZ=off  SenseTotalTorque=off  SenseTotalTorqueX=off  SenseTotalTorqueY=off  SenseTotalTorqueZ=off  CompositeWrenchDir=FollowerOnBase  CompositeWrenchFrame=BaseFrame  EquilibriumPosition=0  EquilibriumPositionUnits=rad  SpringStiffness=0  SpringStiffnessUnits=N*m/rad  DampingCoefficient=0  DampingCoefficientUnits=N*m/(rad/s)  TorqueActuationMode=NoTorque  MotionActuationMode=ComputedMotion  SensePosition=off  SenseVelocity=off  SenseAcceleration=off  SenseTorqueForce=off  PositionTargetSpecify=off  PositionTargetPriority=High  PositionTargetValue=0  PositionTargetValueUnits=deg  VelocityTargetSpecify=off  VelocityTargetPriority=High  VelocityTargetValue=0  VelocityTargetValueUnits=deg/s
  Revolute58 : sm_lib/Joints/Revolute Joint  SenseConstraintForce=off  SenseConstraintForceX=off  SenseConstraintForceY=off  SenseConstraintForceZ=off  SenseConstraintTorque=off  SenseConstraintTorqueX=off  SenseConstraintTorqueY=off  SenseConstraintTorqueZ=off  SenseTotalForce=off  SenseTotalForceX=off  SenseTotalForceY=off  SenseTotalForceZ=off  SenseTotalTorque=off  SenseTotalTorqueX=off  SenseTotalTorqueY=off  SenseTotalTorqueZ=off  CompositeWrenchDir=FollowerOnBase  CompositeWrenchFrame=BaseFrame  EquilibriumPosition=0  EquilibriumPositionUnits=rad  SpringStiffness=0  SpringStiffnessUnits=N*m/rad  DampingCoefficient=0  DampingCoefficientUnits=N*m/(rad/s)  TorqueActuationMode=NoTorque  MotionActuationMode=ComputedMotion  SensePosition=off  SenseVelocity=off  SenseAcceleration=off  SenseTorqueForce=off  PositionTargetSpecify=on  PositionTargetPriority=Low  PositionTargetValue=smiData.RevoluteJoint(687).Rz.Pos  PositionTargetValueUnits=deg  VelocityTargetSpecify=off  VelocityTargetPriority=High  VelocityTargetValue=0  VelocityTargetValueUnits=deg/s
  Revolute59 : sm_lib/Joints/Revolute Joint  SenseConstraintForce=off  SenseConstraintForceX=off  SenseConstraintForceY=off  SenseConstraintForceZ=off  SenseConstraintTorque=off  SenseConstraintTorqueX=off  SenseConstraintTorqueY=off  SenseConstraintTorqueZ=off  SenseTotalForce=off  SenseTotalForceX=off  SenseTotalForceY=off  SenseTotalForceZ=off  SenseTotalTorque=off  SenseTotalTorqueX=off  SenseTotalTorqueY=off  SenseTotalTorqueZ=off  CompositeWrenchDir=FollowerOnBase  CompositeWrenchFrame=BaseFrame  EquilibriumPosition=0  EquilibriumPositionUnits=rad  SpringStiffness=0  SpringStiffnessUnits=N*m/rad  DampingCoefficient=0  DampingCoefficientUnits=N*m/(rad/s)  TorqueActuationMode=NoTorque  MotionActuationMode=ComputedMotion  SensePosition=off  SenseVelocity=off  SenseAcceleration=off  SenseTorqueForce=off  PositionTargetSpecify=on  PositionTargetPriority=Low  PositionTargetValue=smiData.RevoluteJoint(688).Rz.Pos  PositionTargetValueUnits=deg  VelocityTargetSpecify=off  VelocityTargetPriority=High  VelocityTargetValue=0  VelocityTargetValueUnits=deg/s
  Revolute6 : sm_lib/Joints/Revolute Joint  SenseConstraintForce=off  SenseConstraintForceX=off  SenseConstraintForceY=off  SenseConstraintForceZ=off  SenseConstraintTorque=off  SenseConstraintTorqueX=off  SenseConstraintTorqueY=off  SenseConstraintTorqueZ=off  SenseTotalForce=off  SenseTotalForceX=off  SenseTotalForceY=off  SenseTotalForceZ=off  SenseTotalTorque=off  SenseTotalTorqueX=off  SenseTotalTorqueY=off  SenseTotalTorqueZ=off  CompositeWrenchDir=FollowerOnBase  CompositeWrenchFrame=BaseFrame  EquilibriumPosition=0  EquilibriumPositionUnits=rad  SpringStiffness=0  SpringStiffnessUnits=N*m/rad  DampingCoefficient=0  DampingCoefficientUnits=N*m/(rad/s)  TorqueActuationMode=NoTorque  MotionActuationMode=ComputedMotion  SensePosition=off  SenseVelocity=off  SenseAcceleration=off  SenseTorqueForce=off  PositionTargetSpecify=on  PositionTargetPriority=Low  PositionTargetValue=smiData.RevoluteJoint(635).Rz.Pos  PositionTargetValueUnits=deg  VelocityTargetSpecify=off  VelocityTargetPriority=High  VelocityTargetValue=0  VelocityTargetValueUnits=deg/s
  Revolute60 : sm_lib/Joints/Revolute Joint  SenseConstraintForce=off  SenseConstraintForceX=off  SenseConstraintForceY=off  SenseConstraintForceZ=off  SenseConstraintTorque=off  SenseConstraintTorqueX=off  SenseConstraintTorqueY=off  SenseConstraintTorqueZ=off  SenseTotalForce=off  SenseTotalForceX=off  SenseTotalForceY=off  SenseTotalForceZ=off  SenseTotalTorque=off  SenseTotalTorqueX=off  SenseTotalTorqueY=off  SenseTotalTorqueZ=off  CompositeWrenchDir=FollowerOnBase  CompositeWrenchFrame=BaseFrame  EquilibriumPosition=0  EquilibriumPositionUnits=rad  SpringStiffness=0  SpringStiffnessUnits=N*m/rad  DampingCoefficient=0  DampingCoefficientUnits=N*m/(rad/s)  TorqueActuationMode=NoTorque  MotionActuationMode=ComputedMotion  SensePosition=off  SenseVelocity=off  SenseAcceleration=off  SenseTorqueForce=off  PositionTargetSpecify=on  PositionTargetPriority=Low  PositionTargetValue=smiData.RevoluteJoint(689).Rz.Pos  PositionTargetValueUnits=deg  VelocityTargetSpecify=off  VelocityTargetPriority=High  VelocityTargetValue=0  VelocityTargetValueUnits=deg/s
  Revolute61 : sm_lib/Joints/Revolute Joint  SenseConstraintForce=off  SenseConstraintForceX=off  SenseConstraintForceY=off  SenseConstraintForceZ=off  SenseConstraintTorque=off  SenseConstraintTorqueX=off  SenseConstraintTorqueY=off  SenseConstraintTorqueZ=off  SenseTotalForce=off  SenseTotalForceX=off  SenseTotalForceY=off  SenseTotalForceZ=off  SenseTotalTorque=off  SenseTotalTorqueX=off  SenseTotalTorqueY=off  SenseTotalTorqueZ=off  CompositeWrenchDir=FollowerOnBase  CompositeWrenchFrame=BaseFrame  EquilibriumPosition=0  EquilibriumPositionUnits=rad  SpringStiffness=0  SpringStiffnessUnits=N*m/rad  DampingCoefficient=0  DampingCoefficientUnits=N*m/(rad/s)  TorqueActuationMode=NoTorque  MotionActuationMode=ComputedMotion  SensePosition=off  SenseVelocity=off  SenseAcceleration=off  SenseTorqueForce=off  PositionTargetSpecify=on  PositionTargetPriority=Low  PositionTargetValue=smiData.RevoluteJoint(690).Rz.Pos  PositionTargetValueUnits=deg  VelocityTargetSpecify=off  VelocityTargetPriority=High  VelocityTargetValue=0  VelocityTargetValueUnits=deg/s
  Revolute62 : sm_lib/Joints/Revolute Joint  SenseConstraintForce=off  SenseConstraintForceX=off  SenseConstraintForceY=off  SenseConstraintForceZ=off  SenseConstraintTorque=off  SenseConstraintTorqueX=off  SenseConstraintTorqueY=off  SenseConstraintTorqueZ=off  SenseTotalForce=off  SenseTotalForceX=off  SenseTotalForceY=off  SenseTotalForceZ=off  SenseTotalTorque=off  SenseTotalTorqueX=off  SenseTotalTorqueY=off  SenseTotalTorqueZ=off  CompositeWrenchDir=FollowerOnBase  CompositeWrenchFrame=BaseFrame  EquilibriumPosition=0  EquilibriumPositionUnits=rad  SpringStiffness=0  SpringStiffnessUnits=N*m/rad  DampingCoefficient=0  DampingCoefficientUnits=N*m/(rad/s)  TorqueActuationMode=NoTorque  MotionActuationMode=ComputedMotion  SensePosition=off  SenseVelocity=off  SenseAcceleration=off  SenseTorqueForce=off  PositionTargetSpecify=on  PositionTargetPriority=Low  PositionTargetValue=smiData.RevoluteJoint(691).Rz.Pos  PositionTargetValueUnits=deg  VelocityTargetSpecify=off  VelocityTargetPriority=High  VelocityTargetValue=0  VelocityTargetValueUnits=deg/s
  Revolute63 : sm_lib/Joints/Revolute Joint  SenseConstraintForce=off  SenseConstraintForceX=off  SenseConstraintForceY=off  SenseConstraintForceZ=off  SenseConstraintTorque=off  SenseConstraintTorqueX=off  SenseConstraintTorqueY=off  SenseConstraintTorqueZ=off  SenseTotalForce=off  SenseTotalForceX=off  SenseTotalForceY=off  SenseTotalForceZ=off  SenseTotalTorque=off  SenseTotalTorqueX=off  SenseTotalTorqueY=off  SenseTotalTorqueZ=off  CompositeWrenchDir=FollowerOnBase  CompositeWrenchFrame=BaseFrame  EquilibriumPosition=0  EquilibriumPositionUnits=rad  SpringStiffness=0  SpringStiffnessUnits=N*m/rad  DampingCoefficient=0  DampingCoefficientUnits=N*m/(rad/s)  TorqueActuationMode=NoTorque  MotionActuationMode=ComputedMotion  SensePosition=off  SenseVelocity=off  SenseAcceleration=off  SenseTorqueForce=off  PositionTargetSpecify=on  PositionTargetPriority=Low  PositionTargetValue=smiData.RevoluteJoint(692).Rz.Pos  PositionTargetValueUnits=deg  VelocityTargetSpecify=off  VelocityTargetPriority=High  VelocityTargetValue=0  VelocityTargetValueUnits=deg/s
  Revolute64 : sm_lib/Joints/Revolute Joint  SenseConstraintForce=off  SenseConstraintForceX=off  SenseConstraintForceY=off  SenseConstraintForceZ=off  SenseConstraintTorque=off  SenseConstraintTorqueX=off  SenseConstraintTorqueY=off  SenseConstraintTorqueZ=off  SenseTotalForce=off  SenseTotalForceX=off  SenseTotalForceY=off  SenseTotalForceZ=off  SenseTotalTorque=off  SenseTotalTorqueX=off  SenseTotalTorqueY=off  SenseTotalTorqueZ=off  CompositeWrenchDir=FollowerOnBase  CompositeWrenchFrame=BaseFrame  EquilibriumPosition=0  EquilibriumPositionUnits=rad  SpringStiffness=0  SpringStiffnessUnits=N*m/rad  DampingCoefficient=0  DampingCoefficientUnits=N*m/(rad/s)  TorqueActuationMode=NoTorque  MotionActuationMode=ComputedMotion  SensePosition=off  SenseVelocity=off  SenseAcceleration=off  SenseTorqueForce=off  PositionTargetSpecify=on  PositionTargetPriority=Low  PositionTargetValue=smiData.RevoluteJoint(693).Rz.Pos  PositionTargetValueUnits=deg  VelocityTargetSpecify=off  VelocityTargetPriority=High  VelocityTargetValue=0  VelocityTargetValueUnits=deg/s
  Revolute65 : sm_lib/Joints/Revolute Joint  SenseConstraintForce=off  SenseConstraintForceX=off  SenseConstraintForceY=off  SenseConstraintForceZ=off  SenseConstraintTorque=off  SenseConstraintTorqueX=off  SenseConstraintTorqueY=off  SenseConstraintTorqueZ=off  SenseTotalForce=off  SenseTotalForceX=off  SenseTotalForceY=off  SenseTotalForceZ=off  SenseTotalTorque=off  SenseTotalTorqueX=off  SenseTotalTorqueY=off  SenseTotalTorqueZ=off  CompositeWrenchDir=FollowerOnBase  CompositeWrenchFrame=BaseFrame  EquilibriumPosition=0  EquilibriumPositionUnits=rad  SpringStiffness=0  SpringStiffnessUnits=N*m/rad  DampingCoefficient=0  DampingCoefficientUnits=N*m/(rad/s)  TorqueActuationMode=NoTorque  MotionActuationMode=ComputedMotion  SensePosition=off  SenseVelocity=off  SenseAcceleration=off  SenseTorqueForce=off  PositionTargetSpecify=on  PositionTargetPriority=Low  PositionTargetValue=smiData.RevoluteJoint(694).Rz.Pos  PositionTargetValueUnits=deg  VelocityTargetSpecify=off  VelocityTargetPriority=High  VelocityTargetValue=0  VelocityTargetValueUnits=deg/s
  Revolute66 : sm_lib/Joints/Revolute Joint  SenseConstraintForce=off  SenseConstraintForceX=off  SenseConstraintForceY=off  SenseConstraintForceZ=off  SenseConstraintTorque=off  SenseConstraintTorqueX=off  SenseConstraintTorqueY=off  SenseConstraintTorqueZ=off  SenseTotalForce=off  SenseTotalForceX=off  SenseTotalForceY=off  SenseTotalForceZ=off  SenseTotalTorque=off  SenseTotalTorqueX=off  SenseTotalTorqueY=off  SenseTotalTorqueZ=off  CompositeWrenchDir=FollowerOnBase  CompositeWrenchFrame=BaseFrame  EquilibriumPosition=0  EquilibriumPositionUnits=rad  SpringStiffness=0  SpringStiffnessUnits=N*m/rad  DampingCoefficient=0  DampingCoefficientUnits=N*m/(rad/s)  TorqueActuationMode=NoTorque  MotionActuationMode=ComputedMotion  SensePosition=off  SenseVelocity=off  SenseAcceleration=off  SenseTorqueForce=off  PositionTargetSpecify=on  PositionTargetPriority=Low  PositionTargetValue=smiData.RevoluteJoint(695).Rz.Pos  PositionTargetValueUnits=deg  VelocityTargetSpecify=off  VelocityTargetPriority=High  VelocityTargetValue=0  VelocityTargetValueUnits=deg/s
  Revolute67 : sm_lib/Joints/Revolute Joint  SenseConstraintForce=off  SenseConstraintForceX=off  SenseConstraintForceY=off  SenseConstraintForceZ=off  SenseConstraintTorque=off  SenseConstraintTorqueX=off  SenseConstraintTorqueY=off  SenseConstraintTorqueZ=off  SenseTotalForce=off  SenseTotalForceX=off  SenseTotalForceY=off  SenseTotalForceZ=off  SenseTotalTorque=off  SenseTotalTorqueX=off  SenseTotalTorqueY=off  SenseTotalTorqueZ=off  CompositeWrenchDir=FollowerOnBase  CompositeWrenchFrame=BaseFrame  EquilibriumPosition=0  EquilibriumPositionUnits=rad  SpringStiffness=0  SpringStiffnessUnits=N*m/rad  DampingCoefficient=0  DampingCoefficientUnits=N*m/(rad/s)  TorqueActuationMode=NoTorque  MotionActuationMode=ComputedMotion  SensePosition=off  SenseVelocity=off  SenseAcceleration=off  SenseTorqueForce=off  PositionTargetSpecify=on  PositionTargetPriority=Low  PositionTargetValue=smiData.RevoluteJoint(696).Rz.Pos  PositionTargetValueUnits=deg  VelocityTargetSpecify=off  VelocityTargetPriority=High  VelocityTargetValue=0  VelocityTargetValueUnits=deg/s
  Revolute68 : sm_lib/Joints/Revolute Joint  SenseConstraintForce=off  SenseConstraintForceX=off  SenseConstraintForceY=off  SenseConstraintForceZ=off  SenseConstraintTorque=off  SenseConstraintTorqueX=off  SenseConstraintTorqueY=off  SenseConstraintTorqueZ=off  SenseTotalForce=off  SenseTotalForceX=off  SenseTotalForceY=off  SenseTotalForceZ=off  SenseTotalTorque=off  SenseTotalTorqueX=off  SenseTotalTorqueY=off  SenseTotalTorqueZ=off  CompositeWrenchDir=FollowerOnBase  CompositeWrenchFrame=BaseFrame  EquilibriumPosition=0  EquilibriumPositionUnits=rad  SpringStiffness=0  SpringStiffnessUnits=N*m/rad  DampingCoefficient=0  DampingCoefficientUnits=N*m/(rad/s)  TorqueActuationMode=NoTorque  MotionActuationMode=ComputedMotion  SensePosition=off  SenseVelocity=off  SenseAcceleration=off  SenseTorqueForce=off  PositionTargetSpecify=on  PositionTargetPriority=Low  PositionTargetValue=smiData.RevoluteJoint(697).Rz.Pos  PositionTargetValueUnits=deg  VelocityTargetSpecify=off  VelocityTargetPriority=High  VelocityTargetValue=0  VelocityTargetValueUnits=deg/s
  Revolute69 : sm_lib/Joints/Revolute Joint  SenseConstraintForce=off  SenseConstraintForceX=off  SenseConstraintForceY=off  SenseConstraintForceZ=off  SenseConstraintTorque=off  SenseConstraintTorqueX=off  SenseConstraintTorqueY=off  SenseConstraintTorqueZ=off  SenseTotalForce=off  SenseTotalForceX=off  SenseTotalForceY=off  SenseTotalForceZ=off  SenseTotalTorque=off  SenseTotalTorqueX=off  SenseTotalTorqueY=off  SenseTotalTorqueZ=off  CompositeWrenchDir=FollowerOnBase  CompositeWrenchFrame=BaseFrame  EquilibriumPosition=0  EquilibriumPositionUnits=rad  SpringStiffness=0  SpringStiffnessUnits=N*m/rad  DampingCoefficient=0  DampingCoefficientUnits=N*m/(rad/s)  TorqueActuationMode=NoTorque  MotionActuationMode=ComputedMotion  SensePosition=off  SenseVelocity=off  SenseAcceleration=off  SenseTorqueForce=off  PositionTargetSpecify=on  PositionTargetPriority=Low  PositionTargetValue=smiData.RevoluteJoint(698).Rz.Pos  PositionTargetValueUnits=deg  VelocityTargetSpecify=off  VelocityTargetPriority=High  VelocityTargetValue=0  VelocityTargetValueUnits=deg/s
  Revolute7 : sm_lib/Joints/Revolute Joint  SenseConstraintForce=off  SenseConstraintForceX=off  SenseConstraintForceY=off  SenseConstraintForceZ=off  SenseConstraintTorque=off  SenseConstraintTorqueX=off  SenseConstraintTorqueY=off  SenseConstraintTorqueZ=off  SenseTotalForce=off  SenseTotalForceX=off  SenseTotalForceY=off  SenseTotalForceZ=off  SenseTotalTorque=off  SenseTotalTorqueX=off  SenseTotalTorqueY=off  SenseTotalTorqueZ=off  CompositeWrenchDir=FollowerOnBase  CompositeWrenchFrame=BaseFrame  EquilibriumPosition=0  EquilibriumPositionUnits=rad  SpringStiffness=0  SpringStiffnessUnits=N*m/rad  DampingCoefficient=0  DampingCoefficientUnits=N*m/(rad/s)  TorqueActuationMode=NoTorque  MotionActuationMode=ComputedMotion  SensePosition=off  SenseVelocity=off  SenseAcceleration=off  SenseTorqueForce=off  PositionTargetSpecify=on  PositionTargetPriority=Low  PositionTargetValue=smiData.RevoluteJoint(636).Rz.Pos  PositionTargetValueUnits=deg  VelocityTargetSpecify=off  VelocityTargetPriority=High  VelocityTargetValue=0  VelocityTargetValueUnits=deg/s
  Revolute70 : sm_lib/Joints/Revolute Joint  SenseConstraintForce=off  SenseConstraintForceX=off  SenseConstraintForceY=off  SenseConstraintForceZ=off  SenseConstraintTorque=off  SenseConstraintTorqueX=off  SenseConstraintTorqueY=off  SenseConstraintTorqueZ=off  SenseTotalForce=off  SenseTotalForceX=off  SenseTotalForceY=off  SenseTotalForceZ=off  SenseTotalTorque=off  SenseTotalTorqueX=off  SenseTotalTorqueY=off  SenseTotalTorqueZ=off  CompositeWrenchDir=FollowerOnBase  CompositeWrenchFrame=BaseFrame  EquilibriumPosition=0  EquilibriumPositionUnits=rad  SpringStiffness=0  SpringStiffnessUnits=N*m/rad  DampingCoefficient=0  DampingCoefficientUnits=N*m/(rad/s)  TorqueActuationMode=NoTorque  MotionActuationMode=ComputedMotion  SensePosition=off  SenseVelocity=off  SenseAcceleration=off  SenseTorqueForce=off  PositionTargetSpecify=on  PositionTargetPriority=Low  PositionTargetValue=smiData.RevoluteJoint(699).Rz.Pos  PositionTargetValueUnits=deg  VelocityTargetSpecify=off  VelocityTargetPriority=High  VelocityTargetValue=0  VelocityTargetValueUnits=deg/s
  Revolute71 : sm_lib/Joints/Revolute Joint  SenseConstraintForce=off  SenseConstraintForceX=off  SenseConstraintForceY=off  SenseConstraintForceZ=off  SenseConstraintTorque=off  SenseConstraintTorqueX=off  SenseConstraintTorqueY=off  SenseConstraintTorqueZ=off  SenseTotalForce=off  SenseTotalForceX=off  SenseTotalForceY=off  SenseTotalForceZ=off  SenseTotalTorque=off  SenseTotalTorqueX=off  SenseTotalTorqueY=off  SenseTotalTorqueZ=off  CompositeWrenchDir=FollowerOnBase  CompositeWrenchFrame=BaseFrame  EquilibriumPosition=0  EquilibriumPositionUnits=rad  SpringStiffness=0  SpringStiffnessUnits=N*m/rad  DampingCoefficient=0  DampingCoefficientUnits=N*m/(rad/s)  TorqueActuationMode=NoTorque  MotionActuationMode=ComputedMotion  SensePosition=off  SenseVelocity=off  SenseAcceleration=off  SenseTorqueForce=off  PositionTargetSpecify=on  PositionTargetPriority=Low  PositionTargetValue=smiData.RevoluteJoint(700).Rz.Pos  PositionTargetValueUnits=deg  VelocityTargetSpecify=off  VelocityTargetPriority=High  VelocityTargetValue=0  VelocityTargetValueUnits=deg/s
  Revolute72 : sm_lib/Joints/Revolute Joint  SenseConstraintForce=off  SenseConstraintForceX=off  SenseConstraintForceY=off  SenseConstraintForceZ=off  SenseConstraintTorque=off  SenseConstraintTorqueX=off  SenseConstraintTorqueY=off  SenseConstraintTorqueZ=off  SenseTotalForce=off  SenseTotalForceX=off  SenseTotalForceY=off  SenseTotalForceZ=off  SenseTotalTorque=off  SenseTotalTorqueX=off  SenseTotalTorqueY=off  SenseTotalTorqueZ=off  CompositeWrenchDir=FollowerOnBase  CompositeWrenchFrame=BaseFrame  EquilibriumPosition=0  EquilibriumPositionUnits=rad  SpringStiffness=0  SpringStiffnessUnits=N*m/rad  DampingCoefficient=0  DampingCoefficientUnits=N*m/(rad/s)  TorqueActuationMode=NoTorque  MotionActuationMode=ComputedMotion  SensePosition=off  SenseVelocity=off  SenseAcceleration=off  SenseTorqueForce=off  PositionTargetSpecify=on  PositionTargetPriority=Low  PositionTargetValue=smiData.RevoluteJoint(701).Rz.Pos  PositionTargetValueUnits=deg  VelocityTargetSpecify=off  VelocityTargetPriority=High  VelocityTargetValue=0  VelocityTargetValueUnits=deg/s
  Revolute73 : sm_lib/Joints/Revolute Joint  SenseConstraintForce=off  SenseConstraintForceX=off  SenseConstraintForceY=off  SenseConstraintForceZ=off  SenseConstraintTorque=off  SenseConstraintTorqueX=off  SenseConstraintTorqueY=off  SenseConstraintTorqueZ=off  SenseTotalForce=off  SenseTotalForceX=off  SenseTotalForceY=off  SenseTotalForceZ=off  SenseTotalTorque=off  SenseTotalTorqueX=off  SenseTotalTorqueY=off  SenseTotalTorqueZ=off  CompositeWrenchDir=FollowerOnBase  CompositeWrenchFrame=BaseFrame  EquilibriumPosition=0  EquilibriumPositionUnits=rad  SpringStiffness=0  SpringStiffnessUnits=N*m/rad  DampingCoefficient=0  DampingCoefficientUnits=N*m/(rad/s)  TorqueActuationMode=NoTorque  MotionActuationMode=ComputedMotion  SensePosition=off  SenseVelocity=off  SenseAcceleration=off  SenseTorqueForce=off  PositionTargetSpecify=on  PositionTargetPriority=Low  PositionTargetValue=smiData.RevoluteJoint(702).Rz.Pos  PositionTargetValueUnits=deg  VelocityTargetSpecify=off  VelocityTargetPriority=High  VelocityTargetValue=0  VelocityTargetValueUnits=deg/s
  Revolute74 : sm_lib/Joints/Revolute Joint  SenseConstraintForce=off  SenseConstraintForceX=off  SenseConstraintForceY=off  SenseConstraintForceZ=off  SenseConstraintTorque=off  SenseConstraintTorqueX=off  SenseConstraintTorqueY=off  SenseConstraintTorqueZ=off  SenseTotalForce=off  SenseTotalForceX=off  SenseTotalForceY=off  SenseTotalForceZ=off  SenseTotalTorque=off  SenseTotalTorqueX=off  SenseTotalTorqueY=off  SenseTotalTorqueZ=off  CompositeWrenchDir=FollowerOnBase  CompositeWrenchFrame=BaseFrame  EquilibriumPosition=0  EquilibriumPositionUnits=rad  SpringStiffness=0  SpringStiffnessUnits=N*m/rad  DampingCoefficient=0  DampingCoefficientUnits=N*m/(rad/s)  TorqueActuationMode=NoTorque  MotionActuationMode=ComputedMotion  SensePosition=off  SenseVelocity=off  SenseAcceleration=off  SenseTorqueForce=off  PositionTargetSpecify=on  PositionTargetPriority=Low  PositionTargetValue=smiData.RevoluteJoint(703).Rz.Pos  PositionTargetValueUnits=deg  VelocityTargetSpecify=off  VelocityTargetPriority=High  VelocityTargetValue=0  VelocityTargetValueUnits=deg/s
  Revolute75 : sm_lib/Joints/Revolute Joint  SenseConstraintForce=off  SenseConstraintForceX=off  SenseConstraintForceY=off  SenseConstraintForceZ=off  SenseConstraintTorque=off  SenseConstraintTorqueX=off  SenseConstraintTorqueY=off  SenseConstraintTorqueZ=off  SenseTotalForce=off  SenseTotalForceX=off  SenseTotalForceY=off  SenseTotalForceZ=off  SenseTotalTorque=off  SenseTotalTorqueX=off  SenseTotalTorqueY=off  SenseTotalTorqueZ=off  CompositeWrenchDir=FollowerOnBase  CompositeWrenchFrame=BaseFrame  EquilibriumPosition=0  EquilibriumPositionUnits=rad  SpringStiffness=0  SpringStiffnessUnits=N*m/rad  DampingCoefficient=0  DampingCoefficientUnits=N*m/(rad/s)  TorqueActuationMode=NoTorque  MotionActuationMode=ComputedMotion  SensePosition=off  SenseVelocity=off  SenseAcceleration=off  SenseTorqueForce=off  PositionTargetSpecify=on  PositionTargetPriority=Low  PositionTargetValue=smiData.RevoluteJoint(704).Rz.Pos  PositionTargetValueUnits=deg  VelocityTargetSpecify=off  VelocityTargetPriority=High  VelocityTargetValue=0  VelocityTargetValueUnits=deg/s
  Revolute76 : sm_lib/Joints/Revolute Joint  SenseConstraintForce=off  SenseConstraintForceX=off  SenseConstraintForceY=off  SenseConstraintForceZ=off  SenseConstraintTorque=off  SenseConstraintTorqueX=off  SenseConstraintTorqueY=off  SenseConstraintTorqueZ=off  SenseTotalForce=off  SenseTotalForceX=off  SenseTotalForceY=off  SenseTotalForceZ=off  SenseTotalTorque=off  SenseTotalTorqueX=off  SenseTotalTorqueY=off  SenseTotalTorqueZ=off  CompositeWrenchDir=FollowerOnBase  CompositeWrenchFrame=BaseFrame  EquilibriumPosition=0  EquilibriumPositionUnits=rad  SpringStiffness=0  SpringStiffnessUnits=N*m/rad  DampingCoefficient=0  DampingCoefficientUnits=N*m/(rad/s)  TorqueActuationMode=NoTorque  MotionActuationMode=ComputedMotion  SensePosition=off  SenseVelocity=off  SenseAcceleration=off  SenseTorqueForce=off  PositionTargetSpecify=on  PositionTargetPriority=Low  PositionTargetValue=smiData.RevoluteJoint(705).Rz.Pos  PositionTargetValueUnits=deg  VelocityTargetSpecify=off  VelocityTargetPriority=High  VelocityTargetValue=0  VelocityTargetValueUnits=deg/s
  Revolute77 : sm_lib/Joints/Revolute Joint  SenseConstraintForce=off  SenseConstraintForceX=off  SenseConstraintForceY=off  SenseConstraintForceZ=off  SenseConstraintTorque=off  SenseConstraintTorqueX=off  SenseConstraintTorqueY=off  SenseConstraintTorqueZ=off  SenseTotalForce=off  SenseTotalForceX=off  SenseTotalForceY=off  SenseTotalForceZ=off  SenseTotalTorque=off  SenseTotalTorqueX=off  SenseTotalTorqueY=off  SenseTotalTorqueZ=off  CompositeWrenchDir=FollowerOnBase  CompositeWrenchFrame=BaseFrame  EquilibriumPosition=0  EquilibriumPositionUnits=rad  SpringStiffness=0  SpringStiffnessUnits=N*m/rad  DampingCoefficient=0  DampingCoefficientUnits=N*m/(rad/s)  TorqueActuationMode=NoTorque  MotionActuationMode=ComputedMotion  SensePosition=off  SenseVelocity=off  SenseAcceleration=off  SenseTorqueForce=off  PositionTargetSpecify=on  PositionTargetPriority=Low  PositionTargetValue=smiData.RevoluteJoint(706).Rz.Pos  PositionTargetValueUnits=deg  VelocityTargetSpecify=off  VelocityTargetPriority=High  VelocityTargetValue=0  VelocityTargetValueUnits=deg/s
  Revolute78 : sm_lib/Joints/Revolute Joint  SenseConstraintForce=off  SenseConstraintForceX=off  SenseConstraintForceY=off  SenseConstraintForceZ=off  SenseConstraintTorque=off  SenseConstraintTorqueX=off  SenseConstraintTorqueY=off  SenseConstraintTorqueZ=off  SenseTotalForce=off  SenseTotalForceX=off  SenseTotalForceY=off  SenseTotalForceZ=off  SenseTotalTorque=off  SenseTotalTorqueX=off  SenseTotalTorqueY=off  SenseTotalTorqueZ=off  CompositeWrenchDir=FollowerOnBase  CompositeWrenchFrame=BaseFrame  EquilibriumPosition=0  EquilibriumPositionUnits=rad  SpringStiffness=0  SpringStiffnessUnits=N*m/rad  DampingCoefficient=0  DampingCoefficientUnits=N*m/(rad/s)  TorqueActuationMode=NoTorque  MotionActuationMode=ComputedMotion  SensePosition=off  SenseVelocity=off  SenseAcceleration=off  SenseTorqueForce=off  PositionTargetSpecify=on  PositionTargetPriority=Low  PositionTargetValue=smiData.RevoluteJoint(707).Rz.Pos  PositionTargetValueUnits=deg  VelocityTargetSpecify=off  VelocityTargetPriority=High  VelocityTargetValue=0  VelocityTargetValueUnits=deg/s
  Revolute79 : sm_lib/Joints/Revolute Joint  SenseConstraintForce=off  SenseConstraintForceX=off  SenseConstraintForceY=off  SenseConstraintForceZ=off  SenseConstraintTorque=off  SenseConstraintTorqueX=off  SenseConstraintTorqueY=off  SenseConstraintTorqueZ=off  SenseTotalForce=off  SenseTotalForceX=off  SenseTotalForceY=off  SenseTotalForceZ=off  SenseTotalTorque=off  SenseTotalTorqueX=off  SenseTotalTorqueY=off  SenseTotalTorqueZ=off  CompositeWrenchDir=FollowerOnBase  CompositeWrenchFrame=BaseFrame  EquilibriumPosition=0  EquilibriumPositionUnits=rad  SpringStiffness=0  SpringStiffnessUnits=N*m/rad  DampingCoefficient=0  DampingCoefficientUnits=N*m/(rad/s)  TorqueActuationMode=NoTorque  MotionActuationMode=ComputedMotion  SensePosition=off  SenseVelocity=off  SenseAcceleration=off  SenseTorqueForce=off  PositionTargetSpecify=on  PositionTargetPriority=Low  PositionTargetValue=smiData.RevoluteJoint(708).Rz.Pos  PositionTargetValueUnits=deg  VelocityTargetSpecify=off  VelocityTargetPriority=High  VelocityTargetValue=0  VelocityTargetValueUnits=deg/s
  Revolute8 : sm_lib/Joints/Revolute Joint  SenseConstraintForce=off  SenseConstraintForceX=off  SenseConstraintForceY=off  SenseConstraintForceZ=off  SenseConstraintTorque=off  SenseConstraintTorqueX=off  SenseConstraintTorqueY=off  SenseConstraintTorqueZ=off  SenseTotalForce=off  SenseTotalForceX=off  SenseTotalForceY=off  SenseTotalForceZ=off  SenseTotalTorque=off  SenseTotalTorqueX=off  SenseTotalTorqueY=off  SenseTotalTorqueZ=off  CompositeWrenchDir=FollowerOnBase  CompositeWrenchFrame=BaseFrame  EquilibriumPosition=0  EquilibriumPositionUnits=rad  SpringStiffness=0  SpringStiffnessUnits=N*m/rad  DampingCoefficient=0  DampingCoefficientUnits=N*m/(rad/s)  TorqueActuationMode=NoTorque  MotionActuationMode=ComputedMotion  SensePosition=off  SenseVelocity=off  SenseAcceleration=off  SenseTorqueForce=off  PositionTargetSpecify=on  PositionTargetPriority=Low  PositionTargetValue=smiData.RevoluteJoint(637).Rz.Pos  PositionTargetValueUnits=deg  VelocityTargetSpecify=off  VelocityTargetPriority=High  VelocityTargetValue=0  VelocityTargetValueUnits=deg/s
  Revolute80 : sm_lib/Joints/Revolute Joint  SenseConstraintForce=off  SenseConstraintForceX=off  SenseConstraintForceY=off  SenseConstraintForceZ=off  SenseConstraintTorque=off  SenseConstraintTorqueX=off  SenseConstraintTorqueY=off  SenseConstraintTorqueZ=off  SenseTotalForce=off  SenseTotalForceX=off  SenseTotalForceY=off  SenseTotalForceZ=off  SenseTotalTorque=off  SenseTotalTorqueX=off  SenseTotalTorqueY=off  SenseTotalTorqueZ=off  CompositeWrenchDir=FollowerOnBase  CompositeWrenchFrame=BaseFrame  EquilibriumPosition=0  EquilibriumPositionUnits=rad  SpringStiffness=0  SpringStiffnessUnits=N*m/rad  DampingCoefficient=0  DampingCoefficientUnits=N*m/(rad/s)  TorqueActuationMode=NoTorque  MotionActuationMode=ComputedMotion  SensePosition=off  SenseVelocity=off  SenseAcceleration=off  SenseTorqueForce=off  PositionTargetSpecify=on  PositionTargetPriority=Low  PositionTargetValue=smiData.RevoluteJoint(709).Rz.Pos  PositionTargetValueUnits=deg  VelocityTargetSpecify=off  VelocityTargetPriority=High  VelocityTargetValue=0  VelocityTargetValueUnits=deg/s
  Revolute81 : sm_lib/Joints/Revolute Joint  SenseConstraintForce=off  SenseConstraintForceX=off  SenseConstraintForceY=off  SenseConstraintForceZ=off  SenseConstraintTorque=off  SenseConstraintTorqueX=off  SenseConstraintTorqueY=off  SenseConstraintTorqueZ=off  SenseTotalForce=off  SenseTotalForceX=off  SenseTotalForceY=off  SenseTotalForceZ=off  SenseTotalTorque=off  SenseTotalTorqueX=off  SenseTotalTorqueY=off  SenseTotalTorqueZ=off  CompositeWrenchDir=FollowerOnBase  CompositeWrenchFrame=BaseFrame  EquilibriumPosition=0  EquilibriumPositionUnits=rad  SpringStiffness=0  SpringStiffnessUnits=N*m/rad  DampingCoefficient=0  DampingCoefficientUnits=N*m/(rad/s)  TorqueActuationMode=NoTorque  MotionActuationMode=ComputedMotion  SensePosition=off  SenseVelocity=off  SenseAcceleration=off  SenseTorqueForce=off  PositionTargetSpecify=on  PositionTargetPriority=Low  PositionTargetValue=smiData.RevoluteJoint(710).Rz.Pos  PositionTargetValueUnits=deg  VelocityTargetSpecify=off  VelocityTargetPriority=High  VelocityTargetValue=0  VelocityTargetValueUnits=deg/s
  Revolute82 : sm_lib/Joints/Revolute Joint  SenseConstraintForce=off  SenseConstraintForceX=off  SenseConstraintForceY=off  SenseConstraintForceZ=off  SenseConstraintTorque=off  SenseConstraintTorqueX=off  SenseConstraintTorqueY=off  SenseConstraintTorqueZ=off  SenseTotalForce=off  SenseTotalForceX=off  SenseTotalForceY=off  SenseTotalForceZ=off  SenseTotalTorque=off  SenseTotalTorqueX=off  SenseTotalTorqueY=off  SenseTotalTorqueZ=off  CompositeWrenchDir=FollowerOnBase  CompositeWrenchFrame=BaseFrame  EquilibriumPosition=0  EquilibriumPositionUnits=rad  SpringStiffness=0  SpringStiffnessUnits=N*m/rad  DampingCoefficient=0  DampingCoefficientUnits=N*m/(rad/s)  TorqueActuationMode=NoTorque  MotionActuationMode=ComputedMotion  SensePosition=off  SenseVelocity=off  SenseAcceleration=off  SenseTorqueForce=off  PositionTargetSpecify=on  PositionTargetPriority=Low  PositionTargetValue=smiData.RevoluteJoint(711).Rz.Pos  PositionTargetValueUnits=deg  VelocityTargetSpecify=off  VelocityTargetPriority=High  VelocityTargetValue=0  VelocityTargetValueUnits=deg/s
  Revolute83 : sm_lib/Joints/Revolute Joint  SenseConstraintForce=off  SenseConstraintForceX=off  SenseConstraintForceY=off  SenseConstraintForceZ=off  SenseConstraintTorque=off  SenseConstraintTorqueX=off  SenseConstraintTorqueY=off  SenseConstraintTorqueZ=off  SenseTotalForce=off  SenseTotalForceX=off  SenseTotalForceY=off  SenseTotalForceZ=off  SenseTotalTorque=off  SenseTotalTorqueX=off  SenseTotalTorqueY=off  SenseTotalTorqueZ=off  CompositeWrenchDir=FollowerOnBase  CompositeWrenchFrame=BaseFrame  EquilibriumPosition=0  EquilibriumPositionUnits=rad  SpringStiffness=0  SpringStiffnessUnits=N*m/rad  DampingCoefficient=0  DampingCoefficientUnits=N*m/(rad/s)  TorqueActuationMode=NoTorque  MotionActuationMode=ComputedMotion  SensePosition=off  SenseVelocity=off  SenseAcceleration=off  SenseTorqueForce=off  PositionTargetSpecify=on  PositionTargetPriority=Low  PositionTargetValue=smiData.RevoluteJoint(712).Rz.Pos  PositionTargetValueUnits=deg  VelocityTargetSpecify=off  VelocityTargetPriority=High  VelocityTargetValue=0  VelocityTargetValueUnits=deg/s
  Revolute84 : sm_lib/Joints/Revolute Joint  SenseConstraintForce=off  SenseConstraintForceX=off  SenseConstraintForceY=off  SenseConstraintForceZ=off  SenseConstraintTorque=off  SenseConstraintTorqueX=off  SenseConstraintTorqueY=off  SenseConstraintTorqueZ=off  SenseTotalForce=off  SenseTotalForceX=off  SenseTotalForceY=off  SenseTotalForceZ=off  SenseTotalTorque=off  SenseTotalTorqueX=off  SenseTotalTorqueY=off  SenseTotalTorqueZ=off  CompositeWrenchDir=FollowerOnBase  CompositeWrenchFrame=BaseFrame  EquilibriumPosition=0  EquilibriumPositionUnits=rad  SpringStiffness=0  SpringStiffnessUnits=N*m/rad  DampingCoefficient=0  DampingCoefficientUnits=N*m/(rad/s)  TorqueActuationMode=NoTorque  MotionActuationMode=ComputedMotion  SensePosition=off  SenseVelocity=off  SenseAcceleration=off  SenseTorqueForce=off  PositionTargetSpecify=on  PositionTargetPriority=Low  PositionTargetValue=smiData.RevoluteJoint(713).Rz.Pos  PositionTargetValueUnits=deg  VelocityTargetSpecify=off  VelocityTargetPriority=High  VelocityTargetValue=0  VelocityTargetValueUnits=deg/s
  Revolute85 : sm_lib/Joints/Revolute Joint  SenseConstraintForce=off  SenseConstraintForceX=off  SenseConstraintForceY=off  SenseConstraintForceZ=off  SenseConstraintTorque=off  SenseConstraintTorqueX=off  SenseConstraintTorqueY=off  SenseConstraintTorqueZ=off  SenseTotalForce=off  SenseTotalForceX=off  SenseTotalForceY=off  SenseTotalForceZ=off  SenseTotalTorque=off  SenseTotalTorqueX=off  SenseTotalTorqueY=off  SenseTotalTorqueZ=off  CompositeWrenchDir=FollowerOnBase  CompositeWrenchFrame=BaseFrame  EquilibriumPosition=0  EquilibriumPositionUnits=rad  SpringStiffness=0  SpringStiffnessUnits=N*m/rad  DampingCoefficient=0  DampingCoefficientUnits=N*m/(rad/s)  TorqueActuationMode=NoTorque  MotionActuationMode=ComputedMotion  SensePosition=off  SenseVelocity=off  SenseAcceleration=off  SenseTorqueForce=off  PositionTargetSpecify=on  PositionTargetPriority=Low  PositionTargetValue=smiData.RevoluteJoint(714).Rz.Pos  PositionTargetValueUnits=deg  VelocityTargetSpecify=off  VelocityTargetPriority=High  VelocityTargetValue=0  VelocityTargetValueUnits=deg/s
  Revolute86 : sm_lib/Joints/Revolute Joint  SenseConstraintForce=off  SenseConstraintForceX=off  SenseConstraintForceY=off  SenseConstraintForceZ=off  SenseConstraintTorque=off  SenseConstraintTorqueX=off  SenseConstraintTorqueY=off  SenseConstraintTorqueZ=off  SenseTotalForce=off  SenseTotalForceX=off  SenseTotalForceY=off  SenseTotalForceZ=off  SenseTotalTorque=off  SenseTotalTorqueX=off  SenseTotalTorqueY=off  SenseTotalTorqueZ=off  CompositeWrenchDir=FollowerOnBase  CompositeWrenchFrame=BaseFrame  EquilibriumPosition=0  EquilibriumPositionUnits=rad  SpringStiffness=0  SpringStiffnessUnits=N*m/rad  DampingCoefficient=0  DampingCoefficientUnits=N*m/(rad/s)  TorqueActuationMode=NoTorque  MotionActuationMode=ComputedMotion  SensePosition=off  SenseVelocity=off  SenseAcceleration=off  SenseTorqueForce=off  PositionTargetSpecify=on  PositionTargetPriority=Low  PositionTargetValue=smiData.RevoluteJoint(715).Rz.Pos  PositionTargetValueUnits=deg  VelocityTargetSpecify=off  VelocityTargetPriority=High  VelocityTargetValue=0  VelocityTargetValueUnits=deg/s
  Revolute87 : sm_lib/Joints/Revolute Joint  SenseConstraintForce=off  SenseConstraintForceX=off  SenseConstraintForceY=off  SenseConstraintForceZ=off  SenseConstraintTorque=off  SenseConstraintTorqueX=off  SenseConstraintTorqueY=off  SenseConstraintTorqueZ=off  SenseTotalForce=off  SenseTotalForceX=off  SenseTotalForceY=off  SenseTotalForceZ=off  SenseTotalTorque=off  SenseTotalTorqueX=off  SenseTotalTorqueY=off  SenseTotalTorqueZ=off  CompositeWrenchDir=FollowerOnBase  CompositeWrenchFrame=BaseFrame  EquilibriumPosition=0  EquilibriumPositionUnits=rad  SpringStiffness=0  SpringStiffnessUnits=N*m/rad  DampingCoefficient=0  DampingCoefficientUnits=N*m/(rad/s)  TorqueActuationMode=NoTorque  MotionActuationMode=ComputedMotion  SensePosition=off  SenseVelocity=off  SenseAcceleration=off  SenseTorqueForce=off  PositionTargetSpecify=on  PositionTargetPriority=Low  PositionTargetValue=smiData.RevoluteJoint(716).Rz.Pos  PositionTargetValueUnits=deg  VelocityTargetSpecify=off  VelocityTargetPriority=High  VelocityTargetValue=0  VelocityTargetValueUnits=deg/s
  Revolute88 : sm_lib/Joints/Revolute Joint  SenseConstraintForce=off  SenseConstraintForceX=off  SenseConstraintForceY=off  SenseConstraintForceZ=off  SenseConstraintTorque=off  SenseConstraintTorqueX=off  SenseConstraintTorqueY=off  SenseConstraintTorqueZ=off  SenseTotalForce=off  SenseTotalForceX=off  SenseTotalForceY=off  SenseTotalForceZ=off  SenseTotalTorque=off  SenseTotalTorqueX=off  SenseTotalTorqueY=off  SenseTotalTorqueZ=off  CompositeWrenchDir=FollowerOnBase  CompositeWrenchFrame=BaseFrame  EquilibriumPosition=0  EquilibriumPositionUnits=rad  SpringStiffness=0  SpringStiffnessUnits=N*m/rad  DampingCoefficient=0  DampingCoefficientUnits=N*m/(rad/s)  TorqueActuationMode=NoTorque  MotionActuationMode=ComputedMotion  SensePosition=off  SenseVelocity=off  SenseAcceleration=off  SenseTorqueForce=off  PositionTargetSpecify=on  PositionTargetPriority=Low  PositionTargetValue=smiData.RevoluteJoint(717).Rz.Pos  PositionTargetValueUnits=deg  VelocityTargetSpecify=off  VelocityTargetPriority=High  VelocityTargetValue=0  VelocityTargetValueUnits=deg/s
  Revolute89 : sm_lib/Joints/Revolute Joint  SenseConstraintForce=off  SenseConstraintForceX=off  SenseConstraintForceY=off  SenseConstraintForceZ=off  SenseConstraintTorque=off  SenseConstraintTorqueX=off  SenseConstraintTorqueY=off  SenseConstraintTorqueZ=off  SenseTotalForce=off  SenseTotalForceX=off  SenseTotalForceY=off  SenseTotalForceZ=off  SenseTotalTorque=off  SenseTotalTorqueX=off  SenseTotalTorqueY=off  SenseTotalTorqueZ=off  CompositeWrenchDir=FollowerOnBase  CompositeWrenchFrame=BaseFrame  EquilibriumPosition=0  EquilibriumPositionUnits=rad  SpringStiffness=0  SpringStiffnessUnits=N*m/rad  DampingCoefficient=0  DampingCoefficientUnits=N*m/(rad/s)  TorqueActuationMode=NoTorque  MotionActuationMode=ComputedMotion  SensePosition=off  SenseVelocity=off  SenseAcceleration=off  SenseTorqueForce=off  PositionTargetSpecify=on  PositionTargetPriority=Low  PositionTargetValue=smiData.RevoluteJoint(718).Rz.Pos  PositionTargetValueUnits=deg  VelocityTargetSpecify=off  VelocityTargetPriority=High  VelocityTargetValue=0  VelocityTargetValueUnits=deg/s
  Revolute9 : sm_lib/Joints/Revolute Joint  SenseConstraintForce=off  SenseConstraintForceX=off  SenseConstraintForceY=off  SenseConstraintForceZ=off  SenseConstraintTorque=off  SenseConstraintTorqueX=off  SenseConstraintTorqueY=off  SenseConstraintTorqueZ=off  SenseTotalForce=off  SenseTotalForceX=off  SenseTotalForceY=off  SenseTotalForceZ=off  SenseTotalTorque=off  SenseTotalTorqueX=off  SenseTotalTorqueY=off  SenseTotalTorqueZ=off  CompositeWrenchDir=FollowerOnBase  CompositeWrenchFrame=BaseFrame  EquilibriumPosition=0  EquilibriumPositionUnits=rad  SpringStiffness=0  SpringStiffnessUnits=N*m/rad  DampingCoefficient=0  DampingCoefficientUnits=N*m/(rad/s)  TorqueActuationMode=NoTorque  MotionActuationMode=ComputedMotion  SensePosition=off  SenseVelocity=off  SenseAcceleration=off  SenseTorqueForce=off  PositionTargetSpecify=on  PositionTargetPriority=Low  PositionTargetValue=smiData.RevoluteJoint(638).Rz.Pos  PositionTargetValueUnits=deg  VelocityTargetSpecify=off  VelocityTargetPriority=High  VelocityTargetValue=0  VelocityTargetValueUnits=deg/s
  Revolute90 : sm_lib/Joints/Revolute Joint  SenseConstraintForce=off  SenseConstraintForceX=off  SenseConstraintForceY=off  SenseConstraintForceZ=off  SenseConstraintTorque=off  SenseConstraintTorqueX=off  SenseConstraintTorqueY=off  SenseConstraintTorqueZ=off  SenseTotalForce=off  SenseTotalForceX=off  SenseTotalForceY=off  SenseTotalForceZ=off  SenseTotalTorque=off  SenseTotalTorqueX=off  SenseTotalTorqueY=off  SenseTotalTorqueZ=off  CompositeWrenchDir=FollowerOnBase  CompositeWrenchFrame=BaseFrame  EquilibriumPosition=0  EquilibriumPositionUnits=rad  SpringStiffness=0  SpringStiffnessUnits=N*m/rad  DampingCoefficient=0  DampingCoefficientUnits=N*m/(rad/s)  TorqueActuationMode=NoTorque  MotionActuationMode=ComputedMotion  SensePosition=off  SenseVelocity=off  SenseAcceleration=off  SenseTorqueForce=off  PositionTargetSpecify=on  PositionTargetPriority=Low  PositionTargetValue=smiData.RevoluteJoint(719).Rz.Pos  PositionTargetValueUnits=deg  VelocityTargetSpecify=off  VelocityTargetPriority=High  VelocityTargetValue=0  VelocityTargetValueUnits=deg/s
  Revolute91 : sm_lib/Joints/Revolute Joint  SenseConstraintForce=off  SenseConstraintForceX=off  SenseConstraintForceY=off  SenseConstraintForceZ=off  SenseConstraintTorque=off  SenseConstraintTorqueX=off  SenseConstraintTorqueY=off  SenseConstraintTorqueZ=off  SenseTotalForce=off  SenseTotalForceX=off  SenseTotalForceY=off  SenseTotalForceZ=off  SenseTotalTorque=off  SenseTotalTorqueX=off  SenseTotalTorqueY=off  SenseTotalTorqueZ=off  CompositeWrenchDir=FollowerOnBase  CompositeWrenchFrame=BaseFrame  EquilibriumPosition=0  EquilibriumPositionUnits=rad  SpringStiffness=0  SpringStiffnessUnits=N*m/rad  DampingCoefficient=0  DampingCoefficientUnits=N*m/(rad/s)  TorqueActuationMode=NoTorque  MotionActuationMode=ComputedMotion  SensePosition=off  SenseVelocity=off  SenseAcceleration=off  SenseTorqueForce=off  PositionTargetSpecify=on  PositionTargetPriority=Low  PositionTargetValue=smiData.RevoluteJoint(720).Rz.Pos  PositionTargetValueUnits=deg  VelocityTargetSpecify=off  VelocityTargetPriority=High  VelocityTargetValue=0  VelocityTargetValueUnits=deg/s
  Revolute92 : sm_lib/Joints/Revolute Joint  SenseConstraintForce=off  SenseConstraintForceX=off  SenseConstraintForceY=off  SenseConstraintForceZ=off  SenseConstraintTorque=off  SenseConstraintTorqueX=off  SenseConstraintTorqueY=off  SenseConstraintTorqueZ=off  SenseTotalForce=off  SenseTotalForceX=off  SenseTotalForceY=off  SenseTotalForceZ=off  SenseTotalTorque=off  SenseTotalTorqueX=off  SenseTotalTorqueY=off  SenseTotalTorqueZ=off  CompositeWrenchDir=FollowerOnBase  CompositeWrenchFrame=BaseFrame  EquilibriumPosition=0  EquilibriumPositionUnits=rad  SpringStiffness=0  SpringStiffnessUnits=N*m/rad  DampingCoefficient=0  DampingCoefficientUnits=N*m/(rad/s)  TorqueActuationMode=NoTorque  MotionActuationMode=ComputedMotion  SensePosition=off  SenseVelocity=off  SenseAcceleration=off  SenseTorqueForce=off  PositionTargetSpecify=on  PositionTargetPriority=Low  PositionTargetValue=smiData.RevoluteJoint(721).Rz.Pos  PositionTargetValueUnits=deg  VelocityTargetSpecify=off  VelocityTargetPriority=High  VelocityTargetValue=0  VelocityTargetValueUnits=deg/s
  Revolute93 : sm_lib/Joints/Revolute Joint  SenseConstraintForce=off  SenseConstraintForceX=off  SenseConstraintForceY=off  SenseConstraintForceZ=off  SenseConstraintTorque=off  SenseConstraintTorqueX=off  SenseConstraintTorqueY=off  SenseConstraintTorqueZ=off  SenseTotalForce=off  SenseTotalForceX=off  SenseTotalForceY=off  SenseTotalForceZ=off  SenseTotalTorque=off  SenseTotalTorqueX=off  SenseTotalTorqueY=off  SenseTotalTorqueZ=off  CompositeWrenchDir=FollowerOnBase  CompositeWrenchFrame=BaseFrame  EquilibriumPosition=0  EquilibriumPositionUnits=rad  SpringStiffness=0  SpringStiffnessUnits=N*m/rad  DampingCoefficient=0  DampingCoefficientUnits=N*m/(rad/s)  TorqueActuationMode=NoTorque  MotionActuationMode=ComputedMotion  SensePosition=off  SenseVelocity=off  SenseAcceleration=off  SenseTorqueForce=off  PositionTargetSpecify=on  PositionTargetPriority=Low  PositionTargetValue=smiData.RevoluteJoint(722).Rz.Pos  PositionTargetValueUnits=deg  VelocityTargetSpecify=off  VelocityTargetPriority=High  VelocityTargetValue=0  VelocityTargetValueUnits=deg/s
  Revolute94 : sm_lib/Joints/Revolute Joint  SenseConstraintForce=off  SenseConstraintForceX=off  SenseConstraintForceY=off  SenseConstraintForceZ=off  SenseConstraintTorque=off  SenseConstraintTorqueX=off  SenseConstraintTorqueY=off  SenseConstraintTorqueZ=off  SenseTotalForce=off  SenseTotalForceX=off  SenseTotalForceY=off  SenseTotalForceZ=off  SenseTotalTorque=off  SenseTotalTorqueX=off  SenseTotalTorqueY=off  SenseTotalTorqueZ=off  CompositeWrenchDir=FollowerOnBase  CompositeWrenchFrame=BaseFrame  EquilibriumPosition=0  EquilibriumPositionUnits=rad  SpringStiffness=0  SpringStiffnessUnits=N*m/rad  DampingCoefficient=0  DampingCoefficientUnits=N*m/(rad/s)  TorqueActuationMode=NoTorque  MotionActuationMode=ComputedMotion  SensePosition=off  SenseVelocity=off  SenseAcceleration=off  SenseTorqueForce=off  PositionTargetSpecify=on  PositionTargetPriority=Low  PositionTargetValue=smiData.RevoluteJoint(723).Rz.Pos  PositionTargetValueUnits=deg  VelocityTargetSpecify=off  VelocityTargetPriority=High  VelocityTargetValue=0  VelocityTargetValueUnits=deg/s
  Revolute95 : sm_lib/Joints/Revolute Joint  SenseConstraintForce=off  SenseConstraintForceX=off  SenseConstraintForceY=off  SenseConstraintForceZ=off  SenseConstraintTorque=off  SenseConstraintTorqueX=off  SenseConstraintTorqueY=off  SenseConstraintTorqueZ=off  SenseTotalForce=off  SenseTotalForceX=off  SenseTotalForceY=off  SenseTotalForceZ=off  SenseTotalTorque=off  SenseTotalTorqueX=off  SenseTotalTorqueY=off  SenseTotalTorqueZ=off  CompositeWrenchDir=FollowerOnBase  CompositeWrenchFrame=BaseFrame  EquilibriumPosition=0  EquilibriumPositionUnits=rad  SpringStiffness=0  SpringStiffnessUnits=N*m/rad  DampingCoefficient=0  DampingCoefficientUnits=N*m/(rad/s)  TorqueActuationMode=NoTorque  MotionActuationMode=ComputedMotion  SensePosition=off  SenseVelocity=off  SenseAcceleration=off  SenseTorqueForce=off  PositionTargetSpecify=on  PositionTargetPriority=Low  PositionTargetValue=smiData.RevoluteJoint(724).Rz.Pos  PositionTargetValueUnits=deg  VelocityTargetSpecify=off  VelocityTargetPriority=High  VelocityTargetValue=0  VelocityTargetValueUnits=deg/s
  Revolute96 : sm_lib/Joints/Revolute Joint  SenseConstraintForce=off  SenseConstraintForceX=off  SenseConstraintForceY=off  SenseConstraintForceZ=off  SenseConstraintTorque=off  SenseConstraintTorqueX=off  SenseConstraintTorqueY=off  SenseConstraintTorqueZ=off  SenseTotalForce=off  SenseTotalForceX=off  SenseTotalForceY=off  SenseTotalForceZ=off  SenseTotalTorque=off  SenseTotalTorqueX=off  SenseTotalTorqueY=off  SenseTotalTorqueZ=off  CompositeWrenchDir=FollowerOnBase  CompositeWrenchFrame=BaseFrame  EquilibriumPosition=0  EquilibriumPositionUnits=rad  SpringStiffness=0  SpringStiffnessUnits=N*m/rad  DampingCoefficient=0  DampingCoefficientUnits=N*m/(rad/s)  TorqueActuationMode=NoTorque  MotionActuationMode=ComputedMotion  SensePosition=off  SenseVelocity=off  SenseAcceleration=off  SenseTorqueForce=off  PositionTargetSpecify=on  PositionTargetPriority=Low  PositionTargetValue=smiData.RevoluteJoint(725).Rz.Pos  PositionTargetValueUnits=deg  VelocityTargetSpecify=off  VelocityTargetPriority=High  VelocityTargetValue=0  VelocityTargetValueUnits=deg/s
  Revolute97 : sm_lib/Joints/Revolute Joint  SenseConstraintForce=off  SenseConstraintForceX=off  SenseConstraintForceY=off  SenseConstraintForceZ=off  SenseConstraintTorque=off  SenseConstraintTorqueX=off  SenseConstraintTorqueY=off  SenseConstraintTorqueZ=off  SenseTotalForce=off  SenseTotalForceX=off  SenseTotalForceY=off  SenseTotalForceZ=off  SenseTotalTorque=off  SenseTotalTorqueX=off  SenseTotalTorqueY=off  SenseTotalTorqueZ=off  CompositeWrenchDir=FollowerOnBase  CompositeWrenchFrame=BaseFrame  EquilibriumPosition=0  EquilibriumPositionUnits=rad  SpringStiffness=0  SpringStiffnessUnits=N*m/rad  DampingCoefficient=0  DampingCoefficientUnits=N*m/(rad/s)  TorqueActuationMode=NoTorque  MotionActuationMode=ComputedMotion  SensePosition=off  SenseVelocity=off  SenseAcceleration=off  SenseTorqueForce=off  PositionTargetSpecify=on  PositionTargetPriority=Low  PositionTargetValue=smiData.RevoluteJoint(726).Rz.Pos  PositionTargetValueUnits=deg  VelocityTargetSpecify=off  VelocityTargetPriority=High  VelocityTargetValue=0  VelocityTargetValueUnits=deg/s
  Revolute98 : sm_lib/Joints/Revolute Joint  SenseConstraintForce=off  SenseConstraintForceX=off  SenseConstraintForceY=off  SenseConstraintForceZ=off  SenseConstraintTorque=off  SenseConstraintTorqueX=off  SenseConstraintTorqueY=off  SenseConstraintTorqueZ=off  SenseTotalForce=off  SenseTotalForceX=off  SenseTotalForceY=off  SenseTotalForceZ=off  SenseTotalTorque=off  SenseTotalTorqueX=off  SenseTotalTorqueY=off  SenseTotalTorqueZ=off  CompositeWrenchDir=FollowerOnBase  CompositeWrenchFrame=BaseFrame  EquilibriumPosition=0  EquilibriumPositionUnits=rad  SpringStiffness=0  SpringStiffnessUnits=N*m/rad  DampingCoefficient=0  DampingCoefficientUnits=N*m/(rad/s)  TorqueActuationMode=NoTorque  MotionActuationMode=ComputedMotion  SensePosition=off  SenseVelocity=off  SenseAcceleration=off  SenseTorqueForce=off  PositionTargetSpecify=on  PositionTargetPriority=Low  PositionTargetValue=smiData.RevoluteJoint(727).Rz.Pos  PositionTargetValueUnits=deg  VelocityTargetSpecify=off  VelocityTargetPriority=High  VelocityTargetValue=0  VelocityTargetValueUnits=deg/s
  Revolute99 : sm_lib/Joints/Revolute Joint  SenseConstraintForce=off  SenseConstraintForceX=off  SenseConstraintForceY=off  SenseConstraintForceZ=off  SenseConstraintTorque=off  SenseConstraintTorqueX=off  SenseConstraintTorqueY=off  SenseConstraintTorqueZ=off  SenseTotalForce=off  SenseTotalForceX=off  SenseTotalForceY=off  SenseTotalForceZ=off  SenseTotalTorque=off  SenseTotalTorqueX=off  SenseTotalTorqueY=off  SenseTotalTorqueZ=off  CompositeWrenchDir=FollowerOnBase  CompositeWrenchFrame=BaseFrame  EquilibriumPosition=0  EquilibriumPositionUnits=rad  SpringStiffness=0  SpringStiffnessUnits=N*m/rad  DampingCoefficient=0  DampingCoefficientUnits=N*m/(rad/s)  TorqueActuationMode=NoTorque  MotionActuationMode=ComputedMotion  SensePosition=off  SenseVelocity=off  SenseAcceleration=off  SenseTorqueForce=off  PositionTargetSpecify=on  PositionTargetPriority=Low  PositionTargetValue=smiData.RevoluteJoint(728).Rz.Pos  PositionTargetValueUnits=deg  VelocityTargetSpecify=off  VelocityTargetPriority=High  VelocityTargetValue=0  VelocityTargetValueUnits=deg/s
  SEA_system_1_RIGID : Subsystem
  SEA_system_4_RIGID : Subsystem
  SEA_system_hip_1_RIGID : Subsystem
  beam_filler_1_RIGID : Subsystem
  beam_filler_2_RIGID : Subsystem
  beam_filler_3_RIGID : Subsystem
  beam_filler_4_RIGID : Subsystem
  beam_filler_hip_1_RIGID : Subsystem
  beam_filler_hip_2_RIGID : Subsystem
  bearing_1_RIGID : Subsystem
  bearing_2_RIGID : Subsystem
  bearing_3_RIGID : Subsystem
  bearing_4_RIGID : Subsystem
  bearing_5_RIGID : Subsystem
  bearing_6_RIGID : Subsystem
  hex_bolt_gradeb_iso_145_RIGID : Subsystem
  hex_bolt_gradeb_iso_146_RIGID : Subsystem
  hex_bolt_gradeb_iso_147_RIGID : Subsystem
  hex_bolt_gradeb_iso_148_RIGID : Subsystem
  hex_bolt_gradeb_iso_149_RIGID : Subsystem
  hex_bolt_gradeb_iso_150_RIGID : Subsystem
  hex_bolt_gradeb_iso_151_RIGID : Subsystem
  hex_bolt_gradeb_iso_152_RIGID : Subsystem
  hex_bolt_gradeb_iso_153_RIGID : Subsystem
  hex_bolt_gradeb_iso_154_RIGID : Subsystem
  hex_bolt_gradeb_iso_155_RIGID : Subsystem
  hex_bolt_gradeb_iso_156_RIGID : Subsystem
  hex_bolt_gradeb_iso_157_RIGID : Subsystem
  hex_bolt_gradeb_iso_158_RIGID : Subsystem
  hex_bolt_gradeb_iso_159_RIGID : Subsystem
  hex_bolt_gradeb_iso_160_RIGID : Subsystem
  hex_bolt_gradeb_iso_161_RIGID : Subsystem
  hex_bolt_gradeb_iso_162_RIGID : Subsystem
  hex_bolt_gradeb_iso_163_RIGID : Subsystem
  hex_bolt_gradeb_iso_164_RIGID : Subsystem
  hex_bolt_gradeb_iso_165_RIGID : Subsystem
  hex_bolt_gradeb_iso_166_RIGID : Subsystem
  hex_bolt_gradeb_iso_167_RIGID : Subsystem
  hex_bolt_gradeb_iso_168_RIGID : Subsystem
  hex_bolt_gradeb_iso_169_RIGID : Subsystem
  hex_bolt_gradeb_iso_170_RIGID : Subsystem
  hex_bolt_gradeb_iso_171_RIGID : Subsystem
  hex_bolt_gradeb_iso_172_RIGID : Subsystem
  hex_bolt_gradeb_iso_173_RIGID : Subsystem
  hex_bolt_gradeb_iso_174_RIGID : Subsystem
  hex_bolt_gradeb_iso_175_RIGID : Subsystem
  hex_bolt_gradeb_iso_176_RIGID : Subsystem
  hex_bolt_gradeb_iso_177_RIGID : Subsystem
  hex_bolt_gradeb_iso_178_RIGID : Subsystem
  hex_bolt_gradeb_iso_179_RIGID : Subsystem
  hex_bolt_gradeb_iso_180_RIGID : Subsystem
  hex_bolt_gradeb_iso_181_RIGID : Subsystem
  hex_bolt_gradeb_iso_182_RIGID : Subsystem
  hex_bolt_gradeb_iso_183_RIGID : Subsystem
  hex_bolt_gradeb_iso_184_RIGID : Subsystem
  hex_bolt_gradeb_iso_185_RIGID : Subsystem
  hex_bolt_gradeb_iso_186_RIGID : Subsystem
  hex_bolt_gradeb_iso_187_RIGID : Subsystem
  hex_bolt_gradeb_iso_188_RIGID : Subsystem
  hex_bolt_gradeb_iso_189_RIGID : Subsystem
  hex_bolt_gradeb_iso_190_RIGID : Subsystem
  hex_bolt_gradeb_iso_191_RIGID : Subsystem
  hex_bolt_gradeb_iso_192_RIGID : Subsystem
  hex_bolt_gradeb_iso_193_RIGID : Subsystem
  hex_bolt_gradeb_iso_194_RIGID : Subsystem
  hex_bolt_gradeb_iso_195_RIGID : Subsystem
  hex_bolt_gradeb_iso_196_RIGID : Subsystem
  hex_bolt_gradeb_iso_197_RIGID : Subsystem
  hex_bolt_gradeb_iso_198_RIGID : Subsystem
  hex_bolt_gradeb_iso_199_RIGID : Subsystem
  hex_bolt_gradeb_iso_200_RIGID : Subsystem
  hex_bolt_gradeb_iso_201_RIGID : Subsystem
  hex_bolt_gradeb_iso_202_RIGID : Subsystem
  hex_bolt_gradeb_iso_203_RIGID : Subsystem
  hex_bolt_gradeb_iso_204_RIGID : Subsystem
  hex_bolt_gradeb_iso_206_RIGID : Subsystem
  hex_bolt_gradeb_iso_207_RIGID : Subsystem
  hex_bolt_gradeb_iso_208_RIGID : Subsystem
  hex_bolt_gradeb_iso_209_RIGID : Subsystem
  hex_bolt_gradeb_iso_210_RIGID : Subsystem
  hex_bolt_gradeb_iso_211_RIGID : Subsystem
  hex_bolt_gradeb_iso_212_RIGID : Subsystem
  hex_bolt_gradeb_iso_213_RIGID : Subsystem
  hex_bolt_gradeb_iso_214_RIGID : Subsystem
  hex_bolt_gradeb_iso_215_RIGID : Subsystem
  hex_bolt_gradeb_iso_216_RIGID : Subsystem
  hex_bolt_gradeb_iso_217_RIGID : Subsystem
  hex_bolt_gradeb_iso_218_RIGID : Subsystem
  hex_bolt_gradeb_iso_219_RIGID : Subsystem
  hex_bolt_gradeb_iso_220_RIGID : Subsystem
  hex_bolt_gradeb_iso_221_RIGID : Subsystem
  hex_bolt_gradeb_iso_222_RIGID : Subsystem
  hex_bolt_gradeb_iso_223_RIGID : Subsystem
  hex_bolt_gradeb_iso_224_RIGID : Subsystem
  hex_bolt_gradeb_iso_225_RIGID : Subsystem
  hex_bolt_gradeb_iso_226_RIGID : Subsystem
  hex_bolt_gradeb_iso_227_RIGID : Subsystem
  hex_bolt_gradeb_iso_228_RIGID : Subsystem
  hex_bolt_gradeb_iso_229_RIGID : Subsystem
  hex_bolt_gradeb_iso_230_RIGID : Subsystem
  hex_bolt_gradeb_iso_231_RIGID : Subsystem
  hex_bolt_gradeb_iso_232_RIGID : Subsystem
  hex_bolt_gradeb_iso_233_RIGID : Subsystem
  hex_bolt_gradeb_iso_234_RIGID : Subsystem
  hex_bolt_gradeb_iso_235_RIGID : Subsystem
  hex_bolt_gradeb_iso_236_RIGID : Subsystem
  hex_bolt_gradeb_iso_237_RIGID : Subsystem
  hex_bolt_gradeb_iso_238_RIGID : Subsystem
  hex_bolt_gradeb_iso_239_RIGID : Subsystem
  hex_bolt_gradeb_iso_240_RIGID : Subsystem
  hex_bolt_gradeb_iso_241_RIGID : Subsystem
  hex_bolt_gradeb_iso_243_RIGID : Subsystem
  hex_bolt_gradeb_iso_244_RIGID : Subsystem
  hex_bolt_gradeb_iso_245_RIGID : Subsystem
  hex_bolt_gradeb_iso_246_RIGID : Subsystem
  hex_bolt_gradeb_iso_247_RIGID : Subsystem
  hex_bolt_gradeb_iso_248_RIGID : Subsystem
  hex_bolt_gradeb_iso_249_RIGID : Subsystem
  hex_bolt_gradeb_iso_250_RIGID : Subsystem
  hex_bolt_gradeb_iso_251_RIGID : Subsystem
  hex_bolt_gradeb_iso_252_RIGID : Subsystem
  hex_bolt_gradeb_iso_253_RIGID : Subsystem
  hex_bolt_gradeb_iso_254_RIGID : Subsystem
  hex_bolt_gradeb_iso_255_RIGID : Subsystem
  hex_bolt_gradeb_iso_256_RIGID : Subsystem
  hex_bolt_gradeb_iso_257_RIGID : Subsystem
  hex_bolt_gradeb_iso_258_RIGID : Subsystem
  hex_bolt_gradeb_iso_259_RIGID : Subsystem
  hex_bolt_gradeb_iso_260_RIGID : Subsystem
  hex_bolt_gradeb_iso_261_RIGID : Subsystem
  hex_bolt_gradeb_iso_262_RIGID : Subsystem
  hex_bolt_gradeb_iso_263_RIGID : Subsystem
  hex_bolt_gradeb_iso_264_RIGID : Subsystem
  hex_bolt_gradeb_iso_265_RIGID : Subsystem
  hex_bolt_gradeb_iso_266_RIGID : Subsystem
  hex_bolt_gradeb_iso_267_RIGID : Subsystem
  hex_bolt_gradeb_iso_268_RIGID : Subsystem
  hex_bolt_gradeb_iso_269_RIGID : Subsystem
  hex_bolt_gradeb_iso_270_RIGID : Subsystem
  hex_bolt_gradeb_iso_271_RIGID : Subsystem
  hex_bolt_gradeb_iso_272_RIGID : Subsystem
  hex_bolt_gradeb_iso_273_RIGID : Subsystem
  hex_bolt_gradeb_iso_274_RIGID : Subsystem
  hex_bolt_gradeb_iso_275_RIGID : Subsystem
  hex_bolt_gradeb_iso_276_RIGID : Subsystem
  hex_bolt_gradeb_iso_277_RIGID : Subsystem
  hex_bolt_gradeb_iso_278_RIGID : Subsystem
  hex_nut_style_1_gradeab_iso_145_RIGID : Subsystem
  hex_nut_style_1_gradeab_iso_146_RIGID : Subsystem
  hex_nut_style_1_gradeab_iso_147_RIGID : Subsystem
  hex_nut_style_1_gradeab_iso_150_RIGID : Subsystem
  hex_nut_style_1_gradeab_iso_151_RIGID : Subsystem
  hex_nut_style_1_gradeab_iso_152_RIGID : Subsystem
  hex_nut_style_1_gradeab_iso_153_RIGID : Subsystem
  hex_nut_style_1_gradeab_iso_154_RIGID : Subsystem
  hex_nut_style_1_gradeab_iso_156_RIGID : Subsystem
  hex_nut_style_1_gradeab_iso_158_RIGID : Subsystem
  hex_nut_style_1_gradeab_iso_159_RIGID : Subsystem
  hex_nut_style_1_gradeab_iso_160_RIGID : Subsystem
  hex_nut_style_1_gradeab_iso_161_RIGID : Subsystem
  hex_nut_style_1_gradeab_iso_162_RIGID : Subsystem
  hex_nut_style_1_gradeab_iso_163_RIGID : Subsystem
  hex_nut_style_1_gradeab_iso_164_RIGID : Subsystem
  hex_nut_style_1_gradeab_iso_165_RIGID : Subsystem
  hex_nut_style_1_gradeab_iso_166_RIGID : Subsystem
  hex_nut_style_1_gradeab_iso_167_RIGID : Subsystem
  hex_nut_style_1_gradeab_iso_168_RIGID : Subsystem
  hex_nut_style_1_gradeab_iso_169_RIGID : Subsystem
  hex_nut_style_1_gradeab_iso_170_RIGID : Subsystem
  hex_nut_style_1_gradeab_iso_171_RIGID : Subsystem
  hex_nut_style_1_gradeab_iso_172_RIGID : Subsystem
  hex_nut_style_1_gradeab_iso_173_RIGID : Subsystem
  hex_nut_style_1_gradeab_iso_174_RIGID : Subsystem
  hex_nut_style_1_gradeab_iso_175_RIGID : Subsystem
  hex_nut_style_1_gradeab_iso_176_RIGID : Subsystem
  hex_nut_style_1_gradeab_iso_177_RIGID : Subsystem
  hex_nut_style_1_gradeab_iso_178_RIGID : Subsystem
  hex_nut_style_1_gradeab_iso_179_RIGID : Subsystem
  hex_nut_style_1_gradeab_iso_180_RIGID : Subsystem
  hex_nut_style_1_gradeab_iso_181_RIGID : Subsystem
  hex_nut_style_1_gradeab_iso_182_RIGID : Subsystem
  hex_nut_style_1_gradeab_iso_183_RIGID : Subsystem
  hex_nut_style_1_gradeab_iso_184_RIGID : Subsystem
  hex_nut_style_1_gradeab_iso_185_RIGID : Subsystem
  hex_nut_style_1_gradeab_iso_186_RIGID : Subsystem
  hex_nut_style_1_gradeab_iso_187_RIGID : Subsystem
  hex_nut_style_1_gradeab_iso_188_RIGID : Subsystem
  hex_nut_style_1_gradeab_iso_189_RIGID : Subsystem
  hex_nut_style_1_gradeab_iso_190_RIGID : Subsystem
  hex_nut_style_1_gradeab_iso_191_RIGID : Subsystem
  hex_nut_style_1_gradeab_iso_192_RIGID : Subsystem
  hex_nut_style_1_gradeab_iso_193_RIGID : Subsystem
  hex_nut_style_1_gradeab_iso_194_RIGID : Subsystem
  hex_nut_style_1_gradeab_iso_195_RIGID : Subsystem
  hex_nut_style_1_gradeab_iso_196_RIGID : Subsystem
  hex_nut_style_1_gradeab_iso_197_RIGID : Subsystem
  hex_nut_style_1_gradeab_iso_198_RIGID : Subsystem
  hex_nut_style_1_gradeab_iso_199_RIGID : Subsystem
  hex_nut_style_1_gradeab_iso_200_RIGID : Subsystem
  hex_nut_style_1_gradeab_iso_201_RIGID : Subsystem
  hex_nut_style_1_gradeab_iso_202_RIGID : Subsystem
  hex_nut_style_1_gradeab_iso_203_RIGID : Subsystem
  hex_nut_style_1_gradeab_iso_204_RIGID : Subsystem
  hex_nut_style_1_gradeab_iso_205_RIGID : Subsystem
  hex_nut_style_1_gradeab_iso_206_RIGID : Subsystem
  hex_nut_style_1_gradeab_iso_207_RIGID : Subsystem
  hex_nut_style_1_gradeab_iso_208_RIGID : Subsystem
  hex_nut_style_1_gradeab_iso_209_RIGID : Subsystem
  hex_nut_style_1_gradeab_iso_210_RIGID : Subsystem
  hex_nut_style_1_gradeab_iso_211_RIGID : Subsystem
  hex_nut_style_1_gradeab_iso_212_RIGID : Subsystem
  hex_nut_style_1_gradeab_iso_213_RIGID : Subsystem
  hex_nut_style_1_gradeab_iso_214_RIGID : Subsystem
  hex_nut_style_1_gradeab_iso_215_RIGID : Subsystem
  hex_nut_style_1_gradeab_iso_216_RIGID : Subsystem
  hex_nut_style_1_gradeab_iso_217_RIGID : Subsystem
  hex_nut_style_1_gradeab_iso_218_RIGID : Subsystem
  hex_nut_style_1_gradeab_iso_219_RIGID : Subsystem
  hex_nut_style_1_gradeab_iso_220_RIGID : Subsystem
  hex_nut_style_1_gradeab_iso_222_RIGID : Subsystem
  hex_nut_style_1_gradeab_iso_223_RIGID : Subsystem
  hex_nut_style_1_gradeab_iso_224_RIGID : Subsystem
  hex_nut_style_1_gradeab_iso_225_RIGID : Subsystem
  hex_nut_style_1_gradeab_iso_226_RIGID : Subsystem
  hex_nut_style_1_gradeab_iso_227_RIGID : Subsystem
  hex_nut_style_1_gradeab_iso_228_RIGID : Subsystem
  hex_nut_style_1_gradeab_iso_229_RIGID : Subsystem
  hex_nut_style_1_gradeab_iso_230_RIGID : Subsystem
  hex_nut_style_1_gradeab_iso_231_RIGID : Subsystem
  hex_nut_style_1_gradeab_iso_232_RIGID : Subsystem
  hex_nut_style_1_gradeab_iso_233_RIGID : Subsystem
  hex_nut_style_1_gradeab_iso_234_RIGID : Subsystem
  hex_nut_style_1_gradeab_iso_235_RIGID : Subsystem
  hex_nut_style_1_gradeab_iso_237_RIGID : Subsystem
  hex_nut_style_1_gradeab_iso_238_RIGID : Subsystem
  hex_nut_style_1_gradeab_iso_239_RIGID : Subsystem
  hex_nut_style_1_gradeab_iso_240_RIGID : Subsystem
  hex_nut_style_1_gradeab_iso_241_RIGID : Subsystem
  hex_nut_style_1_gradeab_iso_242_RIGID : Subsystem
  hex_nut_style_1_gradeab_iso_243_RIGID : Subsystem
  hex_nut_style_1_gradeab_iso_244_RIGID : Subsystem
  hex_nut_style_1_gradeab_iso_247_RIGID : Subsystem
  hex_nut_style_1_gradeab_iso_248_RIGID : Subsystem
  hex_nut_style_1_gradeab_iso_249_RIGID : Subsystem
  hex_nut_style_1_gradeab_iso_250_RIGID : Subsystem
  hex_nut_style_1_gradeab_iso_251_RIGID : Subsystem
  hex_nut_style_1_gradeab_iso_252_RIGID : Subsystem
  hex_nut_style_1_gradeab_iso_253_RIGID : Subsystem
  hex_nut_style_1_gradeab_iso_254_RIGID : Subsystem
  hex_nut_style_1_gradeab_iso_255_RIGID : Subsystem
  hex_nut_style_1_gradeab_iso_256_RIGID : Subsystem
  hex_nut_style_1_gradeab_iso_257_RIGID : Subsystem
  hex_nut_style_1_gradeab_iso_258_RIGID : Subsystem
  hex_nut_style_1_gradeab_iso_259_RIGID : Subsystem
  hex_nut_style_1_gradeab_iso_260_RIGID : Subsystem
  hex_nut_style_1_gradeab_iso_261_RIGID : Subsystem
  hex_nut_style_1_gradeab_iso_262_RIGID : Subsystem
  hex_nut_style_1_gradeab_iso_263_RIGID : Subsystem
  hex_nut_style_1_gradeab_iso_264_RIGID : Subsystem
  hex_nut_style_1_gradeab_iso_265_RIGID : Subsystem
  hex_nut_style_1_gradeab_iso_266_RIGID : Subsystem
  hex_nut_style_1_gradeab_iso_267_RIGID : Subsystem
  hex_nut_style_1_gradeab_iso_268_RIGID : Subsystem
  hex_nut_style_1_gradeab_iso_269_RIGID : Subsystem
  hex_nut_style_1_gradeab_iso_270_RIGID : Subsystem
  hex_nut_style_1_gradeab_iso_271_RIGID : Subsystem
  hex_nut_style_1_gradeab_iso_272_RIGID : Subsystem
  hex_nut_style_1_gradeab_iso_273_RIGID : Subsystem
  hex_nut_style_1_gradeab_iso_274_RIGID : Subsystem
  hex_nut_style_1_gradeab_iso_275_RIGID : Subsystem
  hex_nut_style_1_gradeab_iso_276_RIGID : Subsystem
  hex_nut_style_1_gradeab_iso_277_RIGID : Subsystem
  hex_nut_style_1_gradeab_iso_278_RIGID : Subsystem
  hex_nut_style_1_gradeab_iso_279_RIGID : Subsystem
  hex_nut_style_1_gradeab_iso_280_RIGID : Subsystem
  hex_nut_style_1_gradeab_iso_281_RIGID : Subsystem
  hex_nut_style_1_gradeab_iso_282_RIGID : Subsystem
  hex_nut_style_1_gradeab_iso_283_RIGID : Subsystem
  hex_nut_style_1_gradeab_iso_284_RIGID : Subsystem
  hip_1_RIGID : Subsystem
  hip_joint_casin_1_RIGID : Subsystem
  hip_joint_casin_2_RIGID : Subsystem
  "leftLegController " : Subsystem
  lower_leg_main_1_RIGID : Subsystem
  motor_axle_1_RIGID : Subsystem
  motor_axle_2_RIGID : Subsystem
  motor_axle_3_RIGID : Subsystem
  motor_body_1_RIGID : Subsystem
  motor_body_2_RIGID : Subsystem
  motor_body_3_RIGID : Subsystem
  upper_leg_cap_10_RIGID : Subsystem
  upper_leg_cap_11_RIGID : Subsystem
  upper_leg_cap_12_RIGID : Subsystem
  upper_leg_cap_13_RIGID : Subsystem
  upper_leg_cap_14_RIGID : Subsystem
  upper_leg_cap_15_RIGID : Subsystem
  upper_leg_cap_16_RIGID : Subsystem
  upper_leg_cap_17_RIGID : Subsystem
  upper_leg_cap_18_RIGID : Subsystem
  upper_leg_cap_1_RIGID : Subsystem
  upper_leg_cap_2_RIGID : Subsystem
  upper_leg_cap_3_RIGID : Subsystem
  upper_leg_cap_4_RIGID : Subsystem
  upper_leg_cap_5_RIGID : Subsystem
  upper_leg_cap_6_RIGID : Subsystem
  upper_leg_cap_7_RIGID : Subsystem
  upper_leg_cap_8_RIGID : Subsystem
  upper_leg_cap_9_RIGID : Subsystem
  upper_leg_casin_2_RIGID : Subsystem
  upper_leg_casin_3_RIGID : Subsystem
  upper_leg_casin_4_RIGID : Subsystem
  upper_leg_casin_5_RIGID : Subsystem
  upper_leg_casin_6_RIGID : Subsystem
  upper_leg_casin_7_RIGID : Subsystem
  upperleg_1_RIGID : Subsystem
  F : PMIOPort  Port=1  Side=Left
  F1 : PMIOPort  Port=2  Side=Left
  connections:
  beam_filler_hip_1_RIGID/LConn1 -- hip_joint_casin_1_RIGID/LConn1
  Revolute/LConn1 -- hip_joint_casin_1_RIGID/RConn14
  Revolute4/RConn1 -- hex_nut_style_1_gradeab_iso_252_RIGID/LConn1
  Planar15/RConn1 -- hex_nut_style_1_gradeab_iso_188_RIGID/LConn2
  Lower_joint_cap_4_RIGID/RConn2 -- Planar16/LConn1
  Planar16/RConn1 -- hex_nut_style_1_gradeab_iso_189_RIGID/LConn2
  Lower_joint_cap_4_RIGID/RConn1 -- Planar17/LConn1
  Planar17/RConn1 -- hex_nut_style_1_gradeab_iso_190_RIGID/LConn2
  Ball_bearing_filler_3_RIGID/LConn1 -- Lower_joint_cap_4_RIGID/LConn1
  Lower_joint_cap_5_RIGID/RConn6 -- Planar18/LConn1
  Planar18/RConn1 -- hex_nut_style_1_gradeab_iso_197_RIGID/LConn2
  Lower_joint_cap_5_RIGID/RConn3 -- Planar19/LConn1
  Planar19/RConn1 -- hex_nut_style_1_gradeab_iso_199_RIGID/LConn2
  Revolute5/LConn1 -- hip_joint_casin_1_RIGID/RConn4
  Lower_joint_cap_5_RIGID/RConn5 -- Planar20/LConn1
  Planar20/RConn1 -- hex_nut_style_1_gradeab_iso_201_RIGID/LConn1
  Lower_joint_cap_5_RIGID/RConn4 -- Planar21/LConn1
  Planar21/RConn1 -- hex_nut_style_1_gradeab_iso_204_RIGID/LConn2
  Lower_joint_cap_5_RIGID/RConn2 -- Planar22/LConn1
  Planar22/RConn1 -- hex_nut_style_1_gradeab_iso_205_RIGID/LConn2
  Lower_joint_cap_5_RIGID/RConn1 -- Planar23/LConn1
  Planar23/RConn1 -- hex_nut_style_1_gradeab_iso_206_RIGID/LConn2
  Ball_bearing_filler_5_RIGID/LConn1 -- Lower_joint_cap_5_RIGID/LConn1
  Lower_joint_cap_6_RIGID/RConn6 -- Revolute32/LConn1
  Revolute5/RConn1 -- hex_nut_style_1_gradeab_iso_253_RIGID/LConn1
  Revolute32/RConn1 -- hex_nut_style_1_gradeab_iso_209_RIGID/LConn1
  Lower_joint_cap_6_RIGID/RConn5 -- Revolute33/LConn1
  Revolute33/RConn1 -- hex_nut_style_1_gradeab_iso_210_RIGID/LConn1
  Lower_joint_cap_6_RIGID/RConn4 -- Revolute34/LConn1
  Revolute34/RConn1 -- hex_nut_style_1_gradeab_iso_211_RIGID/LConn1
  Lower_joint_cap_6_RIGID/RConn3 -- Revolute35/LConn1
  Revolute35/RConn1 -- hex_nut_style_1_gradeab_iso_212_RIGID/LConn1
  Lower_joint_cap_6_RIGID/RConn2 -- Revolute36/LConn1
  Revolute36/RConn1 -- hex_nut_style_1_gradeab_iso_213_RIGID/LConn1
  Lower_joint_cap_6_RIGID/RConn1 -- Revolute37/LConn1
  Revolute6/LConn1 -- hip_joint_casin_1_RIGID/RConn3
  Revolute37/RConn1 -- hex_nut_style_1_gradeab_iso_214_RIGID/LConn1
  Ball_bearing_filler_6_RIGID/LConn1 -- Lower_joint_cap_6_RIGID/LConn1
  Revolute38/LConn1 -- upper_leg_cap_10_RIGID/RConn6
  Revolute38/RConn1 -- hex_nut_style_1_gradeab_iso_175_RIGID/LConn1
  Revolute39/LConn1 -- upper_leg_cap_10_RIGID/RConn5
  Revolute39/RConn1 -- hex_nut_style_1_gradeab_iso_176_RIGID/LConn1
  Revolute40/LConn1 -- upper_leg_cap_10_RIGID/RConn4
  Revolute40/RConn1 -- hex_nut_style_1_gradeab_iso_178_RIGID/LConn1
  Revolute41/LConn1 -- upper_leg_cap_10_RIGID/RConn3
  Revolute41/RConn1 -- hex_nut_style_1_gradeab_iso_179_RIGID/LConn1
  Revolute6/RConn1 -- hex_nut_style_1_gradeab_iso_254_RIGID/LConn1
  Revolute42/LConn1 -- upper_leg_cap_10_RIGID/RConn2
  Revolute42/RConn1 -- hex_nut_style_1_gradeab_iso_182_RIGID/LConn1
  Revolute43/LConn1 -- upper_leg_cap_10_RIGID/RConn1
  Revolute43/RConn1 -- hex_nut_style_1_gradeab_iso_183_RIGID/LConn1
  Ball_bearing_filler_small_4_RIGID/LConn1 -- upper_leg_cap_10_RIGID/LConn1
  upper_leg_cap_11_RIGID/LConn1 -- upper_leg_cap_17_RIGID/LConn1
  Planar24/LConn1 -- bearing_5_RIGID/RConn2
  Planar24/RConn1 -- upper_leg_cap_11_RIGID/LConn3
  Ball_bearing_filler_small_6_RIGID/LConn3 -- upper_leg_cap_11_RIGID/LConn2
  Planar25/LConn1 -- upper_leg_cap_12_RIGID/RConn1
  Revolute7/LConn1 -- hip_joint_casin_1_RIGID/RConn2
  Planar25/RConn1 -- upper_leg_cap_18_RIGID/LConn2
  Planar26/LConn1 -- bearing_6_RIGID/RConn2
  Planar26/RConn1 -- upper_leg_cap_12_RIGID/LConn3
  Ball_bearing_filler_small_5_RIGID/LConn3 -- upper_leg_cap_12_RIGID/LConn1
  Prismatic/LConn1 -- upper_leg_casin_6_RIGID/RConn13
  Prismatic/RConn1 -- upper_leg_cap_12_RIGID/LConn2
  upper_leg_cap_13_RIGID/LConn2 -- upper_leg_casin_7_RIGID/LConn3
  upper_leg_cap_13_RIGID/LConn1 -- upper_leg_cap_1_RIGID/LConn2
  upper_leg_cap_14_RIGID/LConn1 -- upper_leg_casin_2_RIGID/LConn2
  Planar27/LConn1 -- upper_leg_cap_7_RIGID/RConn1
  Revolute7/RConn1 -- hex_bolt_gradeb_iso_212_RIGID/LConn1
  Planar27/RConn1 -- upper_leg_cap_14_RIGID/LConn2
  Revolute44/LConn1 -- upper_leg_casin_4_RIGID/RConn13
  Revolute44/RConn1 -- upper_leg_cap_15_RIGID/LConn1
  Revolute45/LConn1 -- upper_leg_cap_4_RIGID/RConn3
  Revolute45/RConn1 -- upper_leg_cap_15_RIGID/LConn2
  Planar28/LConn1 -- upper_leg_casin_3_RIGID/RConn13
  Planar28/RConn1 -- upper_leg_cap_16_RIGID/LConn2
  upper_leg_cap_16_RIGID/LConn1 -- upper_leg_cap_3_RIGID/LConn2
  Cylindrical/LConn1 -- upper_leg_cap_17_RIGID/RConn1
  Cylindrical/RConn1 -- upper_leg_cap_18_RIGID/LConn3
  Revolute8/LConn1 -- hip_joint_casin_1_RIGID/RConn1
  Revolute46/LConn1 -- upper_leg_casin_5_RIGID/RConn5
  Revolute46/RConn1 -- upper_leg_cap_17_RIGID/LConn2
  upper_leg_cap_18_RIGID/LConn1 -- upper_leg_casin_6_RIGID/LConn2
  Revolute47/LConn1 -- motor_axle_1_RIGID/RConn3
  Revolute47/RConn1 -- motor_body_1_RIGID/LConn1
  Revolute48/LConn1 -- motor_axle_2_RIGID/RConn1
  Revolute48/RConn1 -- motor_body_2_RIGID/LConn2
  Prismatic1/LConn1 -- motor_axle_2_RIGID/RConn2
  Prismatic1/RConn1 -- SEA_system_4_RIGID/LConn1
  Revolute49/LConn1 -- motor_axle_3_RIGID/RConn3
  Revolute8/RConn1 -- hex_bolt_gradeb_iso_213_RIGID/LConn1
  Revolute49/RConn1 -- motor_body_3_RIGID/LConn1
  Prismatic2/LConn1 -- motor_axle_3_RIGID/RConn2
  Prismatic2/RConn1 -- SEA_system_1_RIGID/LConn1
  Revolute50/LConn1 -- bearing_3_RIGID/RConn2
  Lower_joint_casin_1_RIGID/LConn2 -- Revolute50/RConn1
  Lower_joint_casin_1_RIGID/RConn12 -- Planar29/LConn1
  Planar29/RConn1 -- hex_nut_style_1_gradeab_iso_240_RIGID/LConn1
  Lower_joint_casin_1_RIGID/RConn11 -- Planar30/LConn1
  Planar30/RConn1 -- hex_nut_style_1_gradeab_iso_241_RIGID/LConn2
  Lower_joint_casin_1_RIGID/RConn7 -- Planar31/LConn1
  Revolute9/LConn1 -- hip_joint_casin_1_RIGID/RConn13
  Planar31/RConn1 -- hex_nut_style_1_gradeab_iso_242_RIGID/LConn1
  Lower_joint_casin_1_RIGID/RConn5 -- Planar32/LConn1
  Planar32/RConn1 -- hex_nut_style_1_gradeab_iso_243_RIGID/LConn2
  Lower_joint_casin_1_RIGID/RConn4 -- Planar33/LConn1
  Planar33/RConn1 -- hex_nut_style_1_gradeab_iso_244_RIGID/LConn1
  Lower_joint_casin_1_RIGID/RConn9 -- Planar34/LConn1
  Planar34/RConn1 -- hex_nut_style_1_gradeab_iso_248_RIGID/LConn1
  Lower_joint_casin_1_RIGID/RConn3 -- Revolute51/LConn1
  Revolute51/RConn1 -- hex_bolt_gradeb_iso_224_RIGID/LConn1
  Lower_joint_casin_1_RIGID/RConn2 -- Revolute52/LConn1
  Revolute/RConn1 -- bearing_2_RIGID/LConn1
  Revolute9/RConn1 -- hex_bolt_gradeb_iso_214_RIGID/LConn1
  Revolute52/RConn1 -- hex_bolt_gradeb_iso_225_RIGID/LConn1
  Lower_joint_casin_1_RIGID/RConn1 -- Revolute53/LConn1
  Revolute53/RConn1 -- hex_bolt_gradeb_iso_226_RIGID/LConn1
  Lower_joint_casin_1_RIGID/RConn10 -- Revolute54/LConn1
  Revolute54/RConn1 -- hex_bolt_gradeb_iso_227_RIGID/LConn1
  Lower_joint_casin_1_RIGID/RConn8 -- Revolute55/LConn1
  Revolute55/RConn1 -- hex_bolt_gradeb_iso_228_RIGID/LConn1
  Lower_joint_casin_1_RIGID/RConn6 -- Revolute56/LConn1
  Revolute56/RConn1 -- hex_bolt_gradeb_iso_229_RIGID/LConn1
  Lower_joint_casin_2_RIGID/RConn13 -- Revolute57/LConn1
  Revolute10/LConn1 -- hip_joint_casin_1_RIGID/RConn12
  Revolute57/RConn1 -- bearing_4_RIGID/LConn2
  Lower_joint_casin_2_RIGID/RConn12 -- Revolute58/LConn1
  Revolute58/RConn1 -- hex_nut_style_1_gradeab_iso_234_RIGID/LConn1
  Lower_joint_casin_2_RIGID/RConn10 -- Revolute59/LConn1
  Revolute59/RConn1 -- hex_nut_style_1_gradeab_iso_235_RIGID/LConn1
  Lower_joint_casin_2_RIGID/RConn9 -- Revolute60/LConn1
  Revolute60/RConn1 -- hex_nut_style_1_gradeab_iso_237_RIGID/LConn1
  Lower_joint_casin_2_RIGID/RConn7 -- Revolute61/LConn1
  Revolute61/RConn1 -- hex_nut_style_1_gradeab_iso_238_RIGID/LConn1
  Lower_joint_casin_2_RIGID/RConn6 -- Revolute62/LConn1
  Revolute10/RConn1 -- hex_bolt_gradeb_iso_215_RIGID/LConn1
  Revolute62/RConn1 -- hex_nut_style_1_gradeab_iso_239_RIGID/LConn1
  Lower_joint_casin_2_RIGID/RConn5 -- Revolute63/LConn1
  Revolute63/RConn1 -- hex_nut_style_1_gradeab_iso_247_RIGID/LConn1
  Lower_joint_casin_2_RIGID/RConn3 -- Revolute64/LConn1
  Revolute64/RConn1 -- hex_bolt_gradeb_iso_218_RIGID/LConn1
  Lower_joint_casin_2_RIGID/RConn2 -- Revolute65/LConn1
  Revolute65/RConn1 -- hex_bolt_gradeb_iso_219_RIGID/LConn1
  Lower_joint_casin_2_RIGID/RConn1 -- Revolute66/LConn1
  Revolute66/RConn1 -- hex_bolt_gradeb_iso_220_RIGID/LConn1
  Lower_joint_casin_2_RIGID/RConn11 -- Revolute67/LConn1
  Revolute11/LConn1 -- hip_joint_casin_1_RIGID/RConn11
  Revolute67/RConn1 -- hex_bolt_gradeb_iso_221_RIGID/LConn1
  Lower_joint_casin_2_RIGID/RConn8 -- Revolute68/LConn1
  Revolute68/RConn1 -- hex_bolt_gradeb_iso_222_RIGID/LConn1
  Lower_joint_casin_2_RIGID/RConn4 -- Revolute69/LConn1
  Revolute69/RConn1 -- hex_bolt_gradeb_iso_223_RIGID/LConn1
  Lower_joint_casin_3_RIGID/RConn11 -- Revolute70/LConn1
  Revolute70/RConn1 -- bearing_5_RIGID/LConn1
  Lower_joint_casin_3_RIGID/RConn13 -- Planar35/LConn1
  Planar35/RConn1 -- hex_nut_style_1_gradeab_iso_279_RIGID/LConn1
  Lower_joint_casin_3_RIGID/RConn10 -- Planar36/LConn1
  Revolute11/RConn1 -- hex_bolt_gradeb_iso_216_RIGID/LConn1
  Planar36/RConn1 -- hex_nut_style_1_gradeab_iso_280_RIGID/LConn1
  Lower_joint_casin_3_RIGID/RConn12 -- Planar37/LConn1
  Planar37/RConn1 -- hex_nut_style_1_gradeab_iso_281_RIGID/LConn1
  Lower_joint_casin_3_RIGID/RConn7 -- Planar38/LConn1
  Planar38/RConn1 -- hex_nut_style_1_gradeab_iso_282_RIGID/LConn1
  Lower_joint_casin_3_RIGID/RConn5 -- Planar39/LConn1
  Planar39/RConn1 -- hex_nut_style_1_gradeab_iso_283_RIGID/LConn2
  Lower_joint_casin_3_RIGID/RConn4 -- Planar40/LConn1
  Planar40/RConn1 -- hex_nut_style_1_gradeab_iso_284_RIGID/LConn2
  Lower_joint_casin_3_RIGID/RConn3 -- Revolute71/LConn1
  Revolute12/LConn1 -- hip_joint_casin_1_RIGID/RConn10
  Revolute71/RConn1 -- hex_bolt_gradeb_iso_230_RIGID/LConn1
  Lower_joint_casin_3_RIGID/RConn2 -- Revolute72/LConn1
  Revolute72/RConn1 -- hex_bolt_gradeb_iso_231_RIGID/LConn1
  Lower_joint_casin_3_RIGID/RConn1 -- Revolute73/LConn1
  Revolute73/RConn1 -- hex_bolt_gradeb_iso_232_RIGID/LConn1
  Lower_joint_casin_3_RIGID/RConn9 -- Revolute74/LConn1
  Revolute74/RConn1 -- hex_bolt_gradeb_iso_233_RIGID/LConn1
  Lower_joint_casin_3_RIGID/RConn8 -- Revolute75/LConn1
  Revolute75/RConn1 -- hex_bolt_gradeb_iso_234_RIGID/LConn1
  Lower_joint_casin_3_RIGID/RConn6 -- Revolute76/LConn1
  Revolute12/RConn1 -- hex_bolt_gradeb_iso_217_RIGID/LConn1
  Revolute76/RConn1 -- hex_bolt_gradeb_iso_235_RIGID/LConn1
  Revolute77/LConn1 -- bearing_6_RIGID/RConn4
  Lower_joint_casin_5_RIGID/LConn1 -- Revolute77/RConn1
  Lower_joint_casin_5_RIGID/RConn12 -- Revolute78/LConn1
  Revolute78/RConn1 -- hex_nut_style_1_gradeab_iso_273_RIGID/LConn1
  Lower_joint_casin_5_RIGID/RConn8 -- Revolute79/LConn1
  Revolute79/RConn1 -- hex_nut_style_1_gradeab_iso_274_RIGID/LConn1
  Lower_joint_casin_5_RIGID/RConn7 -- Revolute80/LConn1
  Revolute80/RConn1 -- hex_nut_style_1_gradeab_iso_275_RIGID/LConn1
  Lower_joint_casin_5_RIGID/RConn6 -- Revolute81/LConn1
  beam_filler_hip_2_RIGID/LConn1 -- hip_joint_casin_2_RIGID/LConn1
  Revolute81/RConn1 -- hex_nut_style_1_gradeab_iso_276_RIGID/LConn1
  Lower_joint_casin_5_RIGID/RConn5 -- Revolute82/LConn1
  Revolute82/RConn1 -- hex_nut_style_1_gradeab_iso_277_RIGID/LConn1
  Lower_joint_casin_5_RIGID/RConn4 -- Revolute83/LConn1
  Revolute83/RConn1 -- hex_nut_style_1_gradeab_iso_278_RIGID/LConn1
  Lower_joint_casin_5_RIGID/RConn3 -- Revolute84/LConn1
  Revolute84/RConn1 -- hex_bolt_gradeb_iso_236_RIGID/LConn1
  Lower_joint_casin_5_RIGID/RConn2 -- Revolute85/LConn1
  Revolute85/RConn1 -- hex_bolt_gradeb_iso_237_RIGID/LConn1
  Lower_joint_casin_5_RIGID/RConn1 -- Revolute86/LConn1
  Revolute13/LConn1 -- bearing_1_RIGID/RConn1
  Revolute86/RConn1 -- hex_bolt_gradeb_iso_238_RIGID/LConn1
  Lower_joint_casin_5_RIGID/RConn11 -- Revolute87/LConn1
  Revolute87/RConn1 -- hex_bolt_gradeb_iso_239_RIGID/LConn1
  Lower_joint_casin_5_RIGID/RConn10 -- Revolute88/LConn1
  Revolute88/RConn1 -- hex_bolt_gradeb_iso_240_RIGID/LConn1
  Lower_joint_casin_5_RIGID/RConn9 -- Revolute89/LConn1
  Revolute89/RConn1 -- hex_bolt_gradeb_iso_241_RIGID/LConn1
  Cylindrical1/LConn1 -- bearing_1_RIGID/RConn3
  Ball_bearing_filler_small_1_RIGID/LConn2 -- Cylindrical1/RConn1
  Cylindrical2/LConn1 -- bearing_2_RIGID/RConn3
  Revolute13/RConn1 -- hip_joint_casin_2_RIGID/LConn2
  Ball_bearing_filler_small_2_RIGID/LConn2 -- Cylindrical2/RConn1
  Cylindrical3/LConn1 -- bearing_5_RIGID/RConn1
  Ball_bearing_filler_small_6_RIGID/LConn2 -- Cylindrical3/RConn1
  Cylindrical4/LConn1 -- bearing_6_RIGID/RConn1
  Ball_bearing_filler_small_5_RIGID/LConn2 -- Cylindrical4/RConn1
  Rectangular/LConn1 -- SEA_system_4_RIGID/RConn1
  Rectangular/RConn1 -- upperleg_1_RIGID/LConn3
  Revolute90/LConn1 -- upperleg_1_RIGID/RConn16
  Revolute90/RConn1 -- hex_bolt_gradeb_iso_169_RIGID/LConn1
  Revolute91/LConn1 -- upperleg_1_RIGID/RConn14
  Revolute1/LConn1 -- hip_joint_casin_1_RIGID/RConn8
  Planar/LConn1 -- hip_joint_casin_2_RIGID/RConn7
  Revolute91/RConn1 -- hex_bolt_gradeb_iso_170_RIGID/LConn1
  Revolute92/LConn1 -- upperleg_1_RIGID/RConn7
  Revolute92/RConn1 -- hex_bolt_gradeb_iso_171_RIGID/LConn1
  Revolute93/LConn1 -- upperleg_1_RIGID/RConn6
  Revolute93/RConn1 -- hex_bolt_gradeb_iso_172_RIGID/LConn1
  Revolute94/LConn1 -- upperleg_1_RIGID/RConn4
  Revolute94/RConn1 -- hex_bolt_gradeb_iso_173_RIGID/LConn1
  Revolute95/LConn1 -- upperleg_1_RIGID/RConn5
  Revolute95/RConn1 -- hex_bolt_gradeb_iso_174_RIGID/LConn1
  Revolute96/LConn1 -- upperleg_1_RIGID/RConn3
  Planar/RConn1 -- hex_nut_style_1_gradeab_iso_255_RIGID/LConn2
  Revolute96/RConn1 -- hex_bolt_gradeb_iso_175_RIGID/LConn1
  Revolute97/LConn1 -- upperleg_1_RIGID/RConn2
  Revolute97/RConn1 -- hex_bolt_gradeb_iso_176_RIGID/LConn1
  Revolute98/LConn1 -- upperleg_1_RIGID/RConn1
  Revolute98/RConn1 -- hex_bolt_gradeb_iso_177_RIGID/LConn1
  Revolute99/LConn1 -- upperleg_1_RIGID/RConn22
  Revolute99/RConn1 -- hex_bolt_gradeb_iso_178_RIGID/LConn1
  Revolute100/LConn1 -- upperleg_1_RIGID/RConn21
  Revolute100/RConn1 -- hex_bolt_gradeb_iso_179_RIGID/LConn1
  Revolute101/LConn1 -- upperleg_1_RIGID/RConn19
  Planar1/LConn1 -- hip_joint_casin_2_RIGID/RConn5
  Revolute101/RConn1 -- hex_bolt_gradeb_iso_180_RIGID/LConn1
  Revolute102/LConn1 -- upperleg_1_RIGID/RConn25
  Revolute102/RConn1 -- hex_bolt_gradeb_iso_181_RIGID/LConn1
  Revolute103/LConn1 -- upperleg_1_RIGID/RConn23
  Revolute103/RConn1 -- hex_bolt_gradeb_iso_182_RIGID/LConn1
  Revolute104/LConn1 -- upperleg_1_RIGID/RConn18
  Revolute104/RConn1 -- hex_bolt_gradeb_iso_183_RIGID/LConn1
  Revolute105/LConn1 -- upperleg_1_RIGID/RConn24
  Revolute105/RConn1 -- hex_bolt_gradeb_iso_184_RIGID/LConn1
  Revolute106/LConn1 -- upperleg_1_RIGID/RConn20
  Planar1/RConn1 -- hex_nut_style_1_gradeab_iso_256_RIGID/LConn2
  Revolute106/RConn1 -- hex_bolt_gradeb_iso_185_RIGID/LConn1
  Revolute107/LConn1 -- upperleg_1_RIGID/RConn17
  Revolute107/RConn1 -- hex_bolt_gradeb_iso_186_RIGID/LConn1
  Revolute108/LConn1 -- upperleg_1_RIGID/RConn15
  Revolute108/RConn1 -- hex_bolt_gradeb_iso_187_RIGID/LConn1
  Revolute109/LConn1 -- upperleg_1_RIGID/RConn13
  Revolute109/RConn1 -- hex_bolt_gradeb_iso_188_RIGID/LConn1
  Revolute110/LConn1 -- upperleg_1_RIGID/RConn12
  Revolute110/RConn1 -- hex_bolt_gradeb_iso_189_RIGID/LConn1
  Revolute111/LConn1 -- upperleg_1_RIGID/RConn11
  Planar2/LConn1 -- hip_joint_casin_2_RIGID/RConn8
  Revolute111/RConn1 -- hex_bolt_gradeb_iso_190_RIGID/LConn1
  Revolute112/LConn1 -- upperleg_1_RIGID/RConn9
  Revolute112/RConn1 -- hex_bolt_gradeb_iso_191_RIGID/LConn1
  Revolute113/LConn1 -- upperleg_1_RIGID/RConn8
  Revolute113/RConn1 -- hex_bolt_gradeb_iso_192_RIGID/LConn1
  Cylindrical5/LConn1 -- hex_bolt_gradeb_iso_244_RIGID/RConn1
  Cylindrical5/RConn1 -- hex_nut_style_1_gradeab_iso_151_RIGID/LConn2
  Cylindrical6/LConn1 -- hex_bolt_gradeb_iso_245_RIGID/RConn1
  Cylindrical6/RConn1 -- hex_nut_style_1_gradeab_iso_152_RIGID/LConn2
  Cylindrical7/LConn1 -- hex_bolt_gradeb_iso_246_RIGID/RConn1
  Planar2/RConn1 -- hex_nut_style_1_gradeab_iso_257_RIGID/LConn1
  Cylindrical7/RConn1 -- hex_nut_style_1_gradeab_iso_153_RIGID/LConn1
  Cylindrical8/LConn1 -- hex_bolt_gradeb_iso_248_RIGID/RConn1
  Cylindrical8/RConn1 -- hex_nut_style_1_gradeab_iso_154_RIGID/LConn1
  Cylindrical9/LConn1 -- hex_bolt_gradeb_iso_243_RIGID/RConn1
  Cylindrical9/RConn1 -- hex_nut_style_1_gradeab_iso_156_RIGID/LConn2
  Cylindrical10/LConn1 -- hex_bolt_gradeb_iso_247_RIGID/RConn1
  Cylindrical10/RConn1 -- hex_nut_style_1_gradeab_iso_158_RIGID/LConn1
  Cylindrical11/LConn1 -- hex_bolt_gradeb_iso_209_RIGID/RConn1
  Cylindrical11/RConn1 -- hex_nut_style_1_gradeab_iso_161_RIGID/LConn2
  Cylindrical12/LConn1 -- hex_bolt_gradeb_iso_211_RIGID/RConn1
  Planar3/LConn1 -- hip_joint_casin_2_RIGID/RConn3
  Cylindrical12/RConn1 -- hex_nut_style_1_gradeab_iso_162_RIGID/LConn1
  Cylindrical13/LConn1 -- hex_bolt_gradeb_iso_208_RIGID/RConn1
  Cylindrical13/RConn1 -- hex_nut_style_1_gradeab_iso_163_RIGID/LConn2
  Cylindrical14/LConn1 -- hex_bolt_gradeb_iso_249_RIGID/RConn1
  Cylindrical14/RConn1 -- hex_nut_style_1_gradeab_iso_164_RIGID/LConn2
  Cylindrical15/LConn1 -- hex_bolt_gradeb_iso_254_RIGID/RConn1
  Cylindrical15/RConn1 -- hex_nut_style_1_gradeab_iso_165_RIGID/LConn2
  Cylindrical16/LConn1 -- hex_bolt_gradeb_iso_253_RIGID/RConn1
  Cylindrical16/RConn1 -- hex_nut_style_1_gradeab_iso_166_RIGID/LConn1
  Cylindrical17/LConn1 -- hex_bolt_gradeb_iso_210_RIGID/RConn1
  Planar3/RConn1 -- hex_nut_style_1_gradeab_iso_258_RIGID/LConn2
  Cylindrical17/RConn1 -- hex_nut_style_1_gradeab_iso_167_RIGID/LConn1
  Cylindrical18/LConn1 -- hex_bolt_gradeb_iso_252_RIGID/RConn1
  Cylindrical18/RConn1 -- hex_nut_style_1_gradeab_iso_168_RIGID/LConn1
  Cylindrical19/LConn1 -- hex_bolt_gradeb_iso_251_RIGID/RConn1
  Cylindrical19/RConn1 -- hex_nut_style_1_gradeab_iso_169_RIGID/LConn2
  Cylindrical20/LConn1 -- hex_bolt_gradeb_iso_250_RIGID/RConn1
  Cylindrical20/RConn1 -- hex_nut_style_1_gradeab_iso_170_RIGID/LConn2
  Cylindrical21/LConn1 -- hex_bolt_gradeb_iso_206_RIGID/RConn1
  Cylindrical21/RConn1 -- hex_nut_style_1_gradeab_iso_171_RIGID/LConn1
  Cylindrical22/LConn1 -- hex_bolt_gradeb_iso_207_RIGID/RConn1
  Planar4/LConn1 -- hip_joint_casin_2_RIGID/RConn2
  Cylindrical22/RConn1 -- hex_nut_style_1_gradeab_iso_172_RIGID/LConn1
  Cylindrical23/LConn1 -- hex_bolt_gradeb_iso_220_RIGID/RConn1
  Cylindrical23/RConn1 -- hex_nut_style_1_gradeab_iso_185_RIGID/LConn1
  Cylindrical24/LConn1 -- hex_bolt_gradeb_iso_221_RIGID/RConn1
  Cylindrical24/RConn1 -- hex_nut_style_1_gradeab_iso_186_RIGID/LConn2
  Cylindrical25/LConn1 -- hex_bolt_gradeb_iso_222_RIGID/RConn1
  Cylindrical25/RConn1 -- hex_nut_style_1_gradeab_iso_187_RIGID/LConn2
  Cylindrical26/LConn1 -- hex_bolt_gradeb_iso_223_RIGID/RConn1
  Cylindrical26/RConn1 -- hex_nut_style_1_gradeab_iso_188_RIGID/LConn1
  Cylindrical27/LConn1 -- hex_bolt_gradeb_iso_218_RIGID/RConn1
  Planar4/RConn1 -- hex_nut_style_1_gradeab_iso_259_RIGID/LConn2
  Cylindrical27/RConn1 -- hex_nut_style_1_gradeab_iso_189_RIGID/LConn1
  Cylindrical28/LConn1 -- hex_bolt_gradeb_iso_219_RIGID/RConn1
  Cylindrical28/RConn1 -- hex_nut_style_1_gradeab_iso_190_RIGID/LConn1
  Cylindrical29/LConn1 -- hex_bolt_gradeb_iso_257_RIGID/RConn1
  Cylindrical29/RConn1 -- hex_nut_style_1_gradeab_iso_191_RIGID/LConn1
  Cylindrical30/LConn1 -- hex_bolt_gradeb_iso_258_RIGID/RConn1
  Cylindrical30/RConn1 -- hex_nut_style_1_gradeab_iso_192_RIGID/LConn2
  Cylindrical31/LConn1 -- hex_bolt_gradeb_iso_259_RIGID/RConn1
  Cylindrical31/RConn1 -- hex_nut_style_1_gradeab_iso_193_RIGID/LConn2
  Cylindrical32/LConn1 -- hex_bolt_gradeb_iso_260_RIGID/RConn1
  Revolute1/RConn1 -- hex_nut_style_1_gradeab_iso_249_RIGID/LConn1
  Planar5/LConn1 -- hip_joint_casin_2_RIGID/RConn1
  Cylindrical32/RConn1 -- hex_nut_style_1_gradeab_iso_194_RIGID/LConn2
  Cylindrical33/LConn1 -- hex_bolt_gradeb_iso_255_RIGID/RConn1
  Cylindrical33/RConn1 -- hex_nut_style_1_gradeab_iso_195_RIGID/LConn1
  Cylindrical34/LConn1 -- hex_bolt_gradeb_iso_256_RIGID/RConn1
  Cylindrical34/RConn1 -- hex_nut_style_1_gradeab_iso_196_RIGID/LConn1
  Cylindrical35/LConn1 -- hex_bolt_gradeb_iso_235_RIGID/RConn1
  Cylindrical35/RConn1 -- hex_nut_style_1_gradeab_iso_197_RIGID/LConn1
  Cylindrical36/LConn1 -- hex_bolt_gradeb_iso_230_RIGID/RConn1
  Cylindrical36/RConn1 -- hex_nut_style_1_gradeab_iso_199_RIGID/LConn1
  Cylindrical37/LConn1 -- hex_bolt_gradeb_iso_234_RIGID/RConn1
  Planar5/RConn1 -- hex_nut_style_1_gradeab_iso_260_RIGID/LConn2
  Cylindrical37/RConn1 -- hex_nut_style_1_gradeab_iso_201_RIGID/LConn2
  Cylindrical38/LConn1 -- hex_bolt_gradeb_iso_233_RIGID/RConn1
  Cylindrical38/RConn1 -- hex_nut_style_1_gradeab_iso_204_RIGID/LConn1
  Cylindrical39/LConn1 -- hex_bolt_gradeb_iso_232_RIGID/RConn1
  Cylindrical39/RConn1 -- hex_nut_style_1_gradeab_iso_205_RIGID/LConn1
  Cylindrical40/LConn1 -- hex_bolt_gradeb_iso_231_RIGID/RConn1
  Cylindrical40/RConn1 -- hex_nut_style_1_gradeab_iso_206_RIGID/LConn1
  Cylindrical41/LConn1 -- hex_bolt_gradeb_iso_268_RIGID/RConn1
  Cylindrical41/RConn1 -- hex_nut_style_1_gradeab_iso_215_RIGID/LConn2
  Cylindrical42/LConn1 -- hex_bolt_gradeb_iso_267_RIGID/RConn1
  Revolute14/LConn1 -- hip_joint_casin_2_RIGID/RConn6
  Cylindrical42/RConn1 -- hex_nut_style_1_gradeab_iso_216_RIGID/LConn1
  Cylindrical43/LConn1 -- hex_bolt_gradeb_iso_271_RIGID/RConn1
  Cylindrical43/RConn1 -- hex_nut_style_1_gradeab_iso_217_RIGID/LConn2
  Cylindrical44/LConn1 -- hex_bolt_gradeb_iso_272_RIGID/RConn1
  Cylindrical44/RConn1 -- hex_nut_style_1_gradeab_iso_218_RIGID/LConn1
  Cylindrical45/LConn1 -- hex_bolt_gradeb_iso_270_RIGID/RConn1
  Cylindrical45/RConn1 -- hex_nut_style_1_gradeab_iso_219_RIGID/LConn1
  Cylindrical46/LConn1 -- hex_bolt_gradeb_iso_269_RIGID/RConn1
  Cylindrical46/RConn1 -- hex_nut_style_1_gradeab_iso_220_RIGID/LConn2
  Cylindrical47/LConn1 -- hex_bolt_gradeb_iso_160_RIGID/RConn1
  Revolute14/RConn1 -- hex_bolt_gradeb_iso_206_RIGID/LConn1
  Cylindrical47/RConn1 -- hex_nut_style_1_gradeab_iso_222_RIGID/LConn1
  Cylindrical48/LConn1 -- hex_bolt_gradeb_iso_161_RIGID/RConn1
  Cylindrical48/RConn1 -- hex_nut_style_1_gradeab_iso_223_RIGID/LConn1
  Cylindrical49/LConn1 -- hex_bolt_gradeb_iso_162_RIGID/RConn1
  Cylindrical49/RConn1 -- hex_nut_style_1_gradeab_iso_224_RIGID/LConn1
  Cylindrical50/LConn1 -- hex_bolt_gradeb_iso_157_RIGID/RConn1
  Cylindrical50/RConn1 -- hex_nut_style_1_gradeab_iso_225_RIGID/LConn1
  Cylindrical51/LConn1 -- hex_bolt_gradeb_iso_158_RIGID/RConn1
  Cylindrical51/RConn1 -- hex_nut_style_1_gradeab_iso_226_RIGID/LConn1
  Cylindrical52/LConn1 -- hex_bolt_gradeb_iso_159_RIGID/RConn1
  Revolute15/LConn1 -- hip_joint_casin_2_RIGID/RConn4
  Cylindrical52/RConn1 -- hex_nut_style_1_gradeab_iso_227_RIGID/LConn2
  Cylindrical53/LConn1 -- hex_bolt_gradeb_iso_166_RIGID/RConn1
  Cylindrical53/RConn1 -- hex_nut_style_1_gradeab_iso_229_RIGID/LConn1
  Cylindrical54/LConn1 -- hex_bolt_gradeb_iso_171_RIGID/RConn1
  Cylindrical54/RConn1 -- hex_nut_style_1_gradeab_iso_240_RIGID/LConn2
  Cylindrical55/LConn1 -- hex_bolt_gradeb_iso_170_RIGID/RConn1
  Cylindrical55/RConn1 -- hex_nut_style_1_gradeab_iso_241_RIGID/LConn1
  Cylindrical56/LConn1 -- hex_bolt_gradeb_iso_174_RIGID/RConn1
  Cylindrical56/RConn1 -- hex_nut_style_1_gradeab_iso_242_RIGID/LConn2
  Cylindrical57/LConn1 -- hex_bolt_gradeb_iso_173_RIGID/RConn1
  Revolute15/RConn1 -- hex_bolt_gradeb_iso_207_RIGID/LConn1
  Cylindrical57/RConn1 -- hex_nut_style_1_gradeab_iso_243_RIGID/LConn1
  Cylindrical58/LConn1 -- hex_bolt_gradeb_iso_172_RIGID/RConn1
  Cylindrical58/RConn1 -- hex_nut_style_1_gradeab_iso_244_RIGID/LConn2
  Cylindrical59/LConn1 -- hex_bolt_gradeb_iso_169_RIGID/RConn1
  Cylindrical59/RConn1 -- hex_nut_style_1_gradeab_iso_248_RIGID/LConn2
  Cylindrical60/LConn1 -- hex_bolt_gradeb_iso_147_RIGID/RConn1
  Cylindrical60/RConn1 -- hex_nut_style_1_gradeab_iso_255_RIGID/LConn1
  Cylindrical61/LConn1 -- hex_bolt_gradeb_iso_148_RIGID/RConn1
  Cylindrical61/RConn1 -- hex_nut_style_1_gradeab_iso_256_RIGID/LConn1
  Cylindrical62/LConn1 -- hex_bolt_gradeb_iso_146_RIGID/RConn1
  Revolute16/LConn1 -- hip_joint_casin_2_RIGID/RConn13
  Cylindrical62/RConn1 -- hex_nut_style_1_gradeab_iso_257_RIGID/LConn2
  Cylindrical63/LConn1 -- hex_bolt_gradeb_iso_150_RIGID/RConn1
  Cylindrical63/RConn1 -- hex_nut_style_1_gradeab_iso_258_RIGID/LConn1
  Cylindrical64/LConn1 -- hex_bolt_gradeb_iso_149_RIGID/RConn1
  Cylindrical64/RConn1 -- hex_nut_style_1_gradeab_iso_259_RIGID/LConn1
  Cylindrical65/LConn1 -- hex_bolt_gradeb_iso_145_RIGID/RConn1
  Cylindrical65/RConn1 -- hex_nut_style_1_gradeab_iso_260_RIGID/LConn1
  Cylindrical66/LConn1 -- hex_bolt_gradeb_iso_181_RIGID/RConn1
  Cylindrical66/RConn1 -- hex_nut_style_1_gradeab_iso_267_RIGID/LConn2
  Cylindrical67/LConn1 -- hex_bolt_gradeb_iso_184_RIGID/RConn1
  Revolute16/RConn1 -- hex_bolt_gradeb_iso_208_RIGID/LConn1
  Cylindrical67/RConn1 -- hex_nut_style_1_gradeab_iso_268_RIGID/LConn1
  Cylindrical68/LConn1 -- hex_bolt_gradeb_iso_185_RIGID/RConn1
  Cylindrical68/RConn1 -- hex_nut_style_1_gradeab_iso_269_RIGID/LConn1
  Cylindrical69/LConn1 -- hex_bolt_gradeb_iso_186_RIGID/RConn1
  Cylindrical69/RConn1 -- hex_nut_style_1_gradeab_iso_270_RIGID/LConn1
  Cylindrical70/LConn1 -- hex_bolt_gradeb_iso_182_RIGID/RConn1
  Cylindrical70/RConn1 -- hex_nut_style_1_gradeab_iso_271_RIGID/LConn1
  Cylindrical71/LConn1 -- hex_bolt_gradeb_iso_183_RIGID/RConn1
  Cylindrical71/RConn1 -- hex_nut_style_1_gradeab_iso_272_RIGID/LConn1
  Cylindrical72/LConn1 -- hex_bolt_gradeb_iso_195_RIGID/RConn1
  Revolute17/LConn1 -- hip_joint_casin_2_RIGID/RConn12
  Cylindrical72/RConn1 -- hex_nut_style_1_gradeab_iso_279_RIGID/LConn2
  Cylindrical73/LConn1 -- hex_bolt_gradeb_iso_194_RIGID/RConn1
  Cylindrical73/RConn1 -- hex_nut_style_1_gradeab_iso_280_RIGID/LConn2
  Cylindrical74/LConn1 -- hex_bolt_gradeb_iso_193_RIGID/RConn1
  Cylindrical74/RConn1 -- hex_nut_style_1_gradeab_iso_281_RIGID/LConn2
  Cylindrical75/LConn1 -- hex_bolt_gradeb_iso_198_RIGID/RConn1
  Cylindrical75/RConn1 -- hex_nut_style_1_gradeab_iso_282_RIGID/LConn2
  Cylindrical76/LConn1 -- hex_bolt_gradeb_iso_197_RIGID/RConn1
  Cylindrical76/RConn1 -- hex_nut_style_1_gradeab_iso_283_RIGID/LConn1
  Cylindrical77/LConn1 -- hex_bolt_gradeb_iso_196_RIGID/RConn1
  Revolute17/RConn1 -- hex_bolt_gradeb_iso_209_RIGID/LConn1
  Cylindrical77/RConn1 -- hex_nut_style_1_gradeab_iso_284_RIGID/LConn1
  Rectangular1/LConn1 -- SEA_system_1_RIGID/RConn1
  Rectangular1/RConn1 -- lower_leg_main_1_RIGID/LConn2
  Revolute114/LConn1 -- lower_leg_main_1_RIGID/RConn12
  Revolute114/RConn1 -- hex_bolt_gradeb_iso_193_RIGID/LConn1
  Revolute115/LConn1 -- lower_leg_main_1_RIGID/RConn8
  Revolute115/RConn1 -- hex_bolt_gradeb_iso_194_RIGID/LConn1
  Revolute116/LConn1 -- lower_leg_main_1_RIGID/RConn7
  Revolute116/RConn1 -- hex_bolt_gradeb_iso_195_RIGID/LConn1
  Revolute117/LConn1 -- lower_leg_main_1_RIGID/RConn4
  Revolute2/LConn1 -- hip_joint_casin_1_RIGID/RConn7
  Revolute18/LConn1 -- hip_joint_casin_2_RIGID/RConn10
  Revolute117/RConn1 -- hex_bolt_gradeb_iso_196_RIGID/LConn1
  Revolute118/LConn1 -- lower_leg_main_1_RIGID/RConn5
  Revolute118/RConn1 -- hex_bolt_gradeb_iso_197_RIGID/LConn1
  Revolute119/LConn1 -- lower_leg_main_1_RIGID/RConn6
  Revolute119/RConn1 -- hex_bolt_gradeb_iso_198_RIGID/LConn1
  Revolute120/LConn1 -- lower_leg_main_1_RIGID/RConn3
  Revolute120/RConn1 -- hex_bolt_gradeb_iso_199_RIGID/LConn1
  Revolute121/LConn1 -- lower_leg_main_1_RIGID/RConn2
  Revolute121/RConn1 -- hex_bolt_gradeb_iso_200_RIGID/LConn1
  Revolute122/LConn1 -- lower_leg_main_1_RIGID/RConn1
  Revolute18/RConn1 -- hex_bolt_gradeb_iso_210_RIGID/LConn1
  Revolute122/RConn1 -- hex_bolt_gradeb_iso_201_RIGID/LConn1
  Revolute123/LConn1 -- lower_leg_main_1_RIGID/RConn11
  Revolute123/RConn1 -- hex_bolt_gradeb_iso_202_RIGID/LConn1
  Revolute124/LConn1 -- lower_leg_main_1_RIGID/RConn10
  Revolute124/RConn1 -- hex_bolt_gradeb_iso_203_RIGID/LConn1
  Revolute125/LConn1 -- lower_leg_main_1_RIGID/RConn9
  Revolute125/RConn1 -- hex_bolt_gradeb_iso_204_RIGID/LConn1
  Revolute126/LConn1 -- upper_leg_casin_2_RIGID/RConn6
  Revolute126/RConn1 -- hex_bolt_gradeb_iso_243_RIGID/LConn1
  Revolute127/LConn1 -- upper_leg_casin_2_RIGID/RConn7
  Revolute19/LConn1 -- hip_joint_casin_2_RIGID/RConn9
  Revolute127/RConn1 -- hex_bolt_gradeb_iso_244_RIGID/LConn1
  Revolute128/LConn1 -- upper_leg_casin_2_RIGID/RConn5
  Revolute128/RConn1 -- hex_bolt_gradeb_iso_245_RIGID/LConn1
  Revolute129/LConn1 -- upper_leg_casin_2_RIGID/RConn4
  Revolute129/RConn1 -- hex_bolt_gradeb_iso_246_RIGID/LConn1
  Revolute130/LConn1 -- upper_leg_casin_2_RIGID/RConn2
  Revolute130/RConn1 -- hex_bolt_gradeb_iso_247_RIGID/LConn1
  Revolute131/LConn1 -- upper_leg_casin_2_RIGID/RConn1
  Revolute131/RConn1 -- hex_bolt_gradeb_iso_248_RIGID/LConn1
  Prismatic3/LConn1 -- upper_leg_casin_2_RIGID/RConn3
  Revolute19/RConn1 -- hex_bolt_gradeb_iso_211_RIGID/LConn1
  Prismatic3/RConn1 -- upper_leg_cap_7_RIGID/LConn1
  motor_body_2_RIGID/LConn1 -- upper_leg_casin_3_RIGID/LConn3
  Planar41/LConn1 -- upper_leg_casin_3_RIGID/RConn8
  Planar41/RConn1 -- hex_nut_style_1_gradeab_iso_222_RIGID/LConn2
  Planar42/LConn1 -- upper_leg_casin_3_RIGID/RConn7
  Planar42/RConn1 -- hex_nut_style_1_gradeab_iso_223_RIGID/LConn2
  Planar43/LConn1 -- upper_leg_casin_3_RIGID/RConn5
  Planar43/RConn1 -- hex_nut_style_1_gradeab_iso_224_RIGID/LConn2
  Planar44/LConn1 -- upper_leg_casin_3_RIGID/RConn6
  Planar44/RConn1 -- hex_nut_style_1_gradeab_iso_225_RIGID/LConn2
  Lower_joint_cap_1_RIGID/RConn6 -- Revolute20/LConn1
  Planar45/LConn1 -- upper_leg_casin_3_RIGID/RConn3
  Planar45/RConn1 -- hex_nut_style_1_gradeab_iso_226_RIGID/LConn2
  Planar46/LConn1 -- upper_leg_casin_3_RIGID/RConn1
  Planar46/RConn1 -- hex_nut_style_1_gradeab_iso_227_RIGID/LConn1
  Revolute132/LConn1 -- upper_leg_casin_3_RIGID/RConn4
  Revolute132/RConn1 -- hex_bolt_gradeb_iso_261_RIGID/LConn1
  Revolute133/LConn1 -- upper_leg_casin_3_RIGID/RConn2
  Revolute133/RConn1 -- hex_bolt_gradeb_iso_262_RIGID/LConn1
  Revolute134/LConn1 -- upper_leg_casin_3_RIGID/RConn12
  Revolute134/RConn1 -- hex_bolt_gradeb_iso_263_RIGID/LConn1
  Revolute20/RConn1 -- hex_nut_style_1_gradeab_iso_145_RIGID/LConn1
  Revolute135/LConn1 -- upper_leg_casin_3_RIGID/RConn11
  Revolute135/RConn1 -- hex_bolt_gradeb_iso_264_RIGID/LConn1
  Revolute136/LConn1 -- upper_leg_casin_3_RIGID/RConn10
  Revolute136/RConn1 -- hex_bolt_gradeb_iso_265_RIGID/LConn1
  Revolute137/LConn1 -- upper_leg_casin_3_RIGID/RConn9
  Revolute137/RConn1 -- hex_bolt_gradeb_iso_266_RIGID/LConn1
  Prismatic4/LConn1 -- upper_leg_cap_3_RIGID/RConn1
  Prismatic4/RConn1 -- upper_leg_casin_3_RIGID/LConn2
  Revolute138/LConn1 -- upper_leg_casin_4_RIGID/RConn12
  Revolute138/RConn1 -- hex_nut_style_1_gradeab_iso_228_RIGID/LConn1
  Lower_joint_cap_1_RIGID/RConn5 -- Revolute21/LConn1
  Planar47/LConn1 -- upper_leg_casin_4_RIGID/RConn4
  Planar47/RConn1 -- hex_nut_style_1_gradeab_iso_229_RIGID/LConn2
  Revolute139/LConn1 -- upper_leg_casin_4_RIGID/RConn8
  Revolute139/RConn1 -- hex_nut_style_1_gradeab_iso_230_RIGID/LConn1
  Revolute140/LConn1 -- upper_leg_casin_4_RIGID/RConn7
  Revolute140/RConn1 -- hex_nut_style_1_gradeab_iso_231_RIGID/LConn1
  Revolute141/LConn1 -- upper_leg_casin_4_RIGID/RConn6
  Revolute141/RConn1 -- hex_nut_style_1_gradeab_iso_232_RIGID/LConn1
  Revolute142/LConn1 -- upper_leg_casin_4_RIGID/RConn5
  Revolute142/RConn1 -- hex_nut_style_1_gradeab_iso_233_RIGID/LConn1
  Revolute21/RConn1 -- hex_nut_style_1_gradeab_iso_146_RIGID/LConn1
  Revolute143/LConn1 -- upper_leg_casin_4_RIGID/RConn3
